simulink model "Noh_Nofusion"  (R2020b)
settings: Solver=FixedStepAuto  StartTime=0.0  StopTime=Inf  FixedStep=0.01  RelTol=1e-3
PostLoadFcn:
  | if any(exist('dsrtsu_mdlpostloadfcn', 'file') ~= 0), dsrtsu_mdlpostloadfcn('Execute', bdroot); end
InitFcn:
  | , if any(exist('rtifpga_mdlclblib', 'file') ~= 0), rtifpga_mdlclblib('Init', bdroot); end,
  | , if any(exist('dsmpb_private', 'file') ~= 0), dsmpb_private('dsmpb_mdlclblib', 'Init', bdroot); end,
undefined symbols (not defined in the file): ACC_TimeGap_DecSetSwt, ACC_TimeGap_IncSetSwt, AccelPedalPosn, AccelPedalPosnVldty, AccelPedlPosnDiagc, AccPedalOverride, ACU_ShiftInProgress, ADAS_Posn_CurLane, AESSwtReq, ALC_SwtReq, BrkPedalSts, CC_ACC_CANCEL_OFFSwt, CC_ACC_CRUISE_OFFSwt, CC_ACC_DecSetSpd_SetSwt, CC_ACC_IncSetSpd_ResuSwt, CC_ACCSwtErr, CharSpd_ms, CSA_NODE, CURRENT_GEAR, CurrentGearValid, DiscIntNeverNeededParam, DrvDoorSts, DrvSBR, DrvTrqReqOvld, ECMACCInterface, ECMRespACC, ELKSwtReq, EngLimpHomeSts, EngSpd, EngState, EngState_PHEV, EngTrqMaxActSpd, EngTrqMinAct, EPS_DrvInpTrqVal_HighReslolution, EPS_FailSts, EPS_LKATorqOvrlDlvd, EPS_LKATorqOvrlDlvdVld, EPS_LKATrqOvlDlvdSts, EPS_SteerMod, EPS_TrqSnsrSts, EQ4_APPINFO, EQ4_LA_ELEM, EQ4_LA_HDR, EQ4_LAP_ELEM, EQ4_LAP_HDR, EQ4_LH_ELEM, EQ4_LH_HDR, EQ4_LRE_ELEM, EQ4_LRE_HDR, ESS_PedSwtReq, ESS_VehSwtReq, FFogLmpSts_F_Pbox, FLWheelDriveDirection, FLWheelSpd, FrntWiprSwtSts, FrntWshrSwtSts, FRWheelDriveDirection, FRWheelSpd, HazardLmpSwtSts, HCU_AccelPedalPosn_Diag ... (+153)
libraries: simulink x132, dsmpblib x27
(part 1 of 14)
PreSaveFcn:
  | , if any(exist('dsmpb_private', 'file') ~= 0), dsmpb_private('dsmpb_mdlclblib', 'PreSave', bdroot); end,
CloseFcn:
  | , if any(exist('dsmpb_private', 'file') ~= 0), dsmpb_private('dsmpb_mdlclblib', 'Close', bdroot); end,
settings Model: RTICANMMDATA=struct('GeneralSetupData',struct('modelroot','D:\ADAS_Store\Project\adas_project','generalsettings',struct('filesettings',struct('destfolder',struct('Name','RTICANMM_FILES','Check',1),'buildfolder',struct('Name','.','Check',1),'AbsDestfolder',struct('Name','D:\ADAS_Store\Project\adas_project\RTICANMM_FILES'),'AbsBuildfolder',struct('Name','D:\ADAS_Store\Project\adas_project'))),'options',struct('addpaths',1,'rmpaths',1,'addtrcexclusion',false,'cannavigator',struct('checkmonitoring',0),'show_usrtrc',0,'use_usrtrc',0),'advanced',struct('options',ones(1,100)),'MPSetup',{{}},'RTI',struct('Type','DSRT','Ver','4.3','Date','02-May-2020'),'modelname','Noh_Nofusion','block','Noh_Nofusion'))  DSRTSU_INTERNAL_RTIFPGA=160  DSMPB_ID_DATA={'104',struct('BlockId','7cff38d8-8644-4a19-b5e4-5036ee6ea8a9','SignalIds',{{'3bbdea8f-b8ec-442d-8749-62bdfef547b6'}}),'1100',struct('BlockId','4ca9a9d8-d3f0-4675-bdb3-98ae5f57268b','SignalIds',{{'65f8c5f7-e719-4be5-a3cd-3d0a65efbc7c','14567e72-e425-4a19-8f08-ff088e7bc1ec','3e363610-daae-4ac2-937f-50da8a805d2e','fbf30fd1-1576-4ae6-a543-209a9facf6d2','e0c202d0-5fb1-4536-b086-d0c57c194c04','c0e2e943-4026-4c35-9218-a0af2d5b6d57','8bfee92f-2cf6-443b-b155-6a457f2e626f','caf28ac8-b870-4c6f-ae52-cb4984ce6abc','2a387729-dd70-441b-bc6e-f3d93104464f','d8bf82ef-2756-4b2f-8a1b-0b3a0445a133','0e21403a-5d1f-447c-bc7f-b58f25cabe9c'}}),'1101',struct('BlockId','d0076d19-96d3-4a18-af19-060cf9157f7a','SignalIds',{{'14858718-5e5f-4783-86cd-d57dc4407506','82655791-0db2-4bf9-9c4e-8101d6dc3df4','e886bc01-ab1a-41e3-b5b9-381a12da1c74','4ac70ee1-afcd-4eba-b446-b68387f1a31e','689c3bac-1bb7-43b0-9971-a5f6a46937d1','02edd042-c75c-428e-8cab-23306c40c90c','cab918fe-db57-43ed-b49c-d58057f13217','ab72ead8-b72e-4302-85f0-2013a3e14f21','1166ec62-eea0-4cb6-ae80-d5b7b4c4a0fa','34e9efe9-6cdc-4a06-9832-9c921a0545b7','1b7d87ae-63cb-4055-a179-c88df6a6f045','ed32b865-3079-4fbe-b7dd-1824d6a55149','7f30ffb5-df1f-4034-bff0-e6d511eebe1b','728925f6-67a6-4dc4-90ab-4b2ad4c99208','c6bc75cb-b181-461a-a367-6900fcbb88bd','8317a6a6-be88-4f57-8078-4578decf736b','48612be6-51f6-4551-8c7e-832774c8bc67','c595a5d8-d15f-4a1e-9efd-3784581641c2','58310f9b-663a-48bf-ac26-6aa723a8a01e','9fd1b362-1098-47fa-bc3e-5a2e8f5c0c2d','451cead1-5ebd-4ac2-ae12-7fbbcf67bb83','9cb3fe7e-65dd-4c40-8287-015a94f704b5','5bf53764-bace-445f-bcc4-fbe30dae6c62','6da7a470-6ef2-4cdb-a51f-4fae12e7471a','60d3bb74-d0fb-48a1-90d5-057b658358a4','ffa9a598-2281-4998-8615-a5ecc23ded37','f9ab87f2-2869-46a8-ab86-8a97089e9558','5064d5d0-55ce-45eb-a3c8-232eacdd7510','e8f543ad-5b2e-4901-86ca-decafb25c62f','1807255d-94a6-48a3-85be-1315832c545a','824ed113-2f14-401d-b956-a14438369d77','260dd518-87ea-4a3e-a881-228651db4719','f5eff198-1af3-4d0e-999d-0c062aab4917','aede5eb3-92b4-4d5d-8021-6c3b3cb83fe8','61c18043-86bd-4be0-a3d8-a1eb1acd2767','42a66cec-6c0c-4b38-bb08-e9ca357fd7a5','56320901-7f7f-449a-abc2-3a4ba0d3d413','9b34d551-a66b-4913-90f3-07aa90245b9a','015840b8-b6ee-4fd1-8636-bb1d9a643f62','c5d51264-f08a-40eb-b0b1-db8cf68002df','711671d4-3b56-48d1-8d4e-8cacf61b19de','d18da288-82ed-49a3-80b3-cf3efb0c0b6d','96ca03ed-5529-4dff-940a-9c6d805b9ee2','176ffabc-6154-4f92-928c-3b9e74565894','4a60be88-e640-4573-bb9c-5438e25d3f5b','54288b0e-bcf5-44a6-9d9a-742a597fbc71','8a2036ac-ec23-4c1d-baf0-14d0d5705fe0'}}),'1102',struct('BlockId','b1879b78-97ae-49bd-be3e-6dd959ea02d7','SignalIds',{{'b184865a-56b8-4642-a9d9-33e216aa1cc7','4f6803c9-4c49-4c0c-bc6a-4fd056ce5919','d43624c1-2988-4cd3-ba78-7b11552dc0b2','0760b15b-d21c-4d21-9c7e-5c6cc820a731','75084567-158f-40fd-b3ae-c40a485083b4','d0e08f80-8df8-4fba-b874-dd6fafcd2bb0','b17d0cf9-4846-48a1-bb2d-a71384e2d6ff','945bc0e0-d807-499a-9365-7adfd37df6fa','58110f9a-7087-4e44-8b20-a6fe297dcb9d','64f52746-4d34-4424-ae18-4dbc9a56c3c7','587e759c-0ed3-4568-8d4e-c2b8e13bca45','b8fe9749-81d7-4d06-8478-96a34fe63437','ebf5961c-0d94-4ce4-b4db-b7b2833f436c','9089f9e4-396a-4d86-8134-6d3956595bad','693d247e-6854-4426-87f7-c7d1ee9d9c13','c20d448c-b801-4195-814c-f833befdaa99','c06ef1b8-55cd-4c64-bdc9-3d9c76d3d8c6','a9470883-42d0-4499-83e8-b60f7ff939b2'}}),'1103',struct('BlockId','40d30207-c21a-4fe9-89b8-31db2ddfcd24','SignalIds',{{'317f5371-3e40-4468-bdfd-f3a914b09fdd','487dc9a7-f215-4486-8edf-23b26ea9e674','56e2ea18-1796-497f-bfc5-34f8a7a00d06','a8fd35e7-70ab-4cf0-bc17-abccda21b043','712b5988-beb7-4069-9325-ac4d1d105b1c','66ba01a0-0e88-4d3a-9ab0-8823bb2078d0','413426c5-cd8c-4ce7-9f02-6918ae7e5a9b','b324e822-3bc5-4738-a954-9bf60ff29b1e','7901db69-3f11-4cf9-a394-c843afd09e88','480f8adf-d9a2-4f97-8224-e59739a90d13','3628ea91-3224-46aa-ab7f-8b572fef6cbe','d84fb504-f908-419d-85e5-1fc1315e5fac','029ee664-06cb-4483-ae91-26f72088f733','37778ae4-2ffb-44fd-a39e-f60bd25d5ad6','f1854a58-8f08-4c6d-9505-83c95ebb36a7','670ec646-6257-4a76-a5d4-ee226aff6fc6','182a7399-08ac-434c-abd3-5469e8d7dc3c','d7a4aba7-220d-44eb-a78e-488b3b0e7d32','f0b7ec55-592a-4cb0-adc7-ca89299845c0','0e6e96cf-5bcb-426b-a6b6-e45252ca00e4','6fe68ad6-5d89-4ea6-a9cc-e00090ddc430','33f16b3a-8526-4185-8ed1-70240d225458','f7e06676-b4f1-4bd4-831a-a554e14d03fb','9f9edd6d-d0a0-4862-92d3-62b44ec6be06'}}),'1104',struct('BlockId','f96afb62-b232-4875-9f16-8cc66b39bf91','SignalIds',{{'60fdcedf-618c-4398-b64e-96a67d35286a','a5abee4c-7192-4b09-b4cb-6b73a01a8785','80a86882-ad5a-461a-9b39-764b3f3b9edb','f2561c9c-264f-4250-ba14-6de6d6d87bfc','5ca34829-1407-46a5-a499-030ccb73446c','b1a0f660-5421-4458-9b14-058e7b19d0a7','3e082988-6105-4757-8f40-1762abe04838','10eebde5-758a-4a7c-9873-029b28255700','b97055ad-af84-4e89-bbec-8426d6ca24a7','02444ee2-6b2a-4c04-bd69-190353a0c672','6b7e1708-e88f-4ff9-b738-fb06481b8050','a61247de-e6d2-4f0d-914d-644a5fac8733','b186f77e-6eeb-4db4-b5e8-55a5ed49ddae','72fb2380-66d9-4408-a4a6-3fdc4c96a441','4b99d9c7-d0fe-4995-8523-0b8e4e0c1a87','993ca2f1-5b4e-4d93-99cb-7f1614d6bccd','d13b3b17-e0b4-40cb-b556-b5fb395c05e3','2b8d32ce-a89a-4bfb-a484-516ae21f5f89'}}),'1105',struct('BlockId','2680f75a-2b29-4fd2-87b5-3498c9e058a6','SignalIds',{{'faa0ae6e-be86-4564-a94c-27f40175599d','4f865cc3-3da2-416a-a28f-e5f9c3832da3','27d74ed4-a669-4b68-bc5c-8acf4c25a9bb','6dbdc5bd-ee8c-480e-9846-77e86fe90609','1cb076e4-082d-4ab9-a5f3-bee85026cdb8','2110b29f-3627-4de3-9efa-dd3d95b1da54','94a8490f-2016-425c-b913-702d8cf19f01','2f9cbf7d-72a1-4bf3-829f-e3c04433bcc1','7f377641-eb9d-4447-8f07-ba1493fdfcbc','32e0a569-e9c5-4c6c-8bcc-77704a185bd1','1a04a7b1-ae91-43b0-927d-b415b38980ab','572d95be-1870-4610-a1b7-429109650953','d91bea2d-baed-4faa-85ed-9673a90f5781','7261506d-eeaa-4777-9a22-f3e4426f086a','10adf570-39c2-4d90-b43f-c59c3584b59b','517bccf7-ae25-4539-b307-30354d195b17','d19821ad-b439-4876-8f19-0734b541c411','df3325a2-916d-48e6-88ff-3bc27aeac87a','22f6a12f-0e34-4c11-b865-9adaabb8b946','66463846-880e-4cdd-9d21-07899b7873a5','07c9a7e7-e28f-4af9-a08a-92ce9b93897a','022c41ff-3ec9-49d1-bfdd-669fbf64d6b6','f28cb986-d944-4ed6-9920-a833a33fef57','804deebe-207b-40c4-8465-d08574e585e9','f3fa9451-9ed3-45ca-88ff-a23189da5307','a157ade1-4d3e-43dc-a7cc-98106a446eca','4b6854fb-31e3-4b06-8063-ea049aa2ba81','62aabf9d-dda7-47f0-85dc-f3ecfe0f445d','c94a70ec-5bac-41e6-aee8-fbef32666ccf','9b83fe42-6781-4ad1-83d7-7c4a17efa7f3','815b8527-3d8f-4145-830e-a0fadbc05b0a','bcdaa839-c535-4875-8ae2-f2aa8b6736eb','674f33aa-9516-4f07-a049-d932dce3789b','a26426b2-6a16-404a-b705-9b68c0dd7dc7','eee14ca8-254f-4116-8e6f-05e0565bedc9','687f108b-366c-4a46-85ac-ac0bcbe55871','b37c0729-9282-4409-ba52-a7f2a4bc6d51','dd0ddc1f-37ff-47ed-8e5f-c2071c6762d6','1b3a4e79-80d6-4094-86f5-78ecd209e112','2232deaf-fd23-43a6-94d6-be881cb58ed4','2a65d406-ac4b-4e2f-ac3c-a87cba00d8b2'}}),'1433',struct('BlockId','94234e05-19a1-4762-bb7b-0b648db02d71','SignalIds',{{'e8c921a0-45c0-4565-a75f-f1538dace8aa','97da14a3-59c2-4f15-9794-12e20298ad37','993ea120-009c-4d58-b833-f257c1bbe946','b0ce32b7-b1b7-4613-8014-a2b096116a3f','d0bc5c4d-081d-493e-bb0f-3880de0830f4','f577c16d-4f84-464d-bc22-208daba2c996','dd8d90c9-db10-4aee-8f78-aab1d2b07a4d','786cc827-4d3f-4751-8aac-002e08b48fca','3cc83904-5789-4284-8d89-c149abb24041','066cabaf-b5cf-4a22-a486-8d7bf34a30a5','14c931a2-4f8a-4067-a3ab-e1ebb5f58bae','3318169c-4586-48c4-8457-857db8f36c39','afa8f609-89b6-4cf2-8b3b-67301da0d077','db3dccf0-ac50-421f-a652-6186d40f7434','98c83b7e-8f23-48c4-966e-4a54d21b7757','42747761-adf1-4162-a5eb-1d7b1815f06f','f4026a07-0643-41fe-ac5d-129eb617d3bb','a806bbcd-b881-4618-9bc2-15c80f567ed0','dd8efa00-8fe6-472b-b374-365213651d88','17e98c86-4a76-41dc-b5a1-c6f316a60d0d','f2c4471e-757c-4a82-8024-244d60e4eae0','0baafb07-de45-4b4b-a0af-fc29d6b90e2f','7deeb15d-c086-41bc-a56a-2c4b692487f1','2b0e0941-927e-4c06-ab5e-2abe3916fc55','5584579c-2ab8-4aaf-b9f9-629067beb1d1','7936e867-fe88-4af5-b973-84858e665a13','c57a407d-b218-42f5-8846-438e73728874','90881888-af9a-4cc4-a1ae-0ecda3135b42','ec3687ed-f2c9-4806-8c7e-30e4660968c6','d4c236ae-2feb-4f6c-9bb1-7b97a6ed9825','8eea8e37-c910-42dc-a602-5540f6a14377','e9ac2b78-f63e-4fc9-95d9-b858b89e45a9','abb40779-4b61-4ab4-bd71-3a821b717804','7fb27904-ab07-458c-959e-9464df60189e','cdef6a3f-3536-4e6e-a717-ef2141c6625b','7766ce8f-4903-4070-8e33-31e989b0c27b','5ed6d31b-ff27-45e5-80f1-63a2314d3977','703c0186-0353-48e4-9ebe-c7e62be1761c','90e2d2bf-e9a2-4e62-963d-e2118c02d3f0','159e3cc7-cce6-4e38-bcaa-fd58f86ac572','7b2e5dd3-de8c-4c77-a57b-9641b9f21836','0c7c6a3d-5efc-4a2c-8d24-02cdd2042006','379efa5b-3a39-4d46-80ca-c859689c2b8e','f549e28d-aeef-4011-b98d-621e8c092949','a26c273e-3059-4d1c-9ca1-60671908df44','8cfd88fd-e834-4fb3-b7a9-6a942acc2f0d','f5cddd7a-0da6-4742-9f4c-10fbd2b3f6f7','8a39439b-2bf1-4344-9b5f-42eb278b8376','8ccf14d9-6c5a-4163-9001-5177855509b8','f5b88dff-d83a-495f-92eb-bece265ce1e6','9dc0ae1f-9d6d-46e8-8842-1ad9d25be10e','5a77b2d3-cbf8-4b9a-a1aa-23d3a249b441','3bcf1e6e-1d26-4903-a127-764aed52a8c4'}}),'1528',struct('BlockId','d10b6a7e-e28c-4d43-9d3f-8d5c2e8198e6','SignalIds',{{'d97805f0-7d23-4e28-bf97-3f26e24bb340'}}),'185',struct('BlockId','027e024d-1595-40f1-91cc-6eabca2a1c6c','SignalIds',{{'af9ca425-4598-4529-ae3a-7e01afab32e2','5b6a4c10-dcc5-4361-b694-7f13522380cd','328b1ae8-99c0-4358-aa60-26f71449921d','56877a5e-a28c-460d-b602-6169d6e3ea29','ff774db8-82bf-4d5d-af96-834818f3b92b','454bb863-e562-4923-b300-500615260782','a069b205-7781-45e2-8fc6-dbc7346dd223','cdcb80d6-e457-4c10-893c-2087872783e0','6b56bd7e-1102-406b-8d36-39d13718a3c9','254c0b29-47ad-419c-85d7-e9515a2bbc5a','a6c2ea10-dbc8-4b2d-879f-4465f4c97ead','84746e2e-380b-4ef4-a4ee-2f1341934cbc','8a1fcb45-6acd-44a7-ab31-c33169900c5c','1bb09bca-435b-416b-bf20-aa9f8dc89494','d5011b75-efa1-42d0-986e-b3cd336946c1','c50ad309-eea6-40fb-8bb2-c8ca0fd215a4','85488a99-7b3a-49f7-9866-9335aff8292f','1b523a6a-dad5-4454-a82b-427cdad5527a','e3668b27-7252-480d-9bc0-b61d6693a235','cdb3337a-376c-4be9-b00d-011122b2f594','9e493416-6a03-4c36-af69-81d560cc7c26','c974d250-90a0-4162-a8f3-f2bd83b95395','d04338fd-2c1d-44c1-83ef-f5a12be17f66','6b9ced49-9cb6-4a69-955c-e404182980a0','b674ae42-370f-4555-9541-dc621716dd61','9984a409-650d-4478-bb6d-7bc56841d6f8','13af6717-7a51-4ea3-9a56-75b6a52376f8','4e0778bb-f83f-41f0-8d20-f78f6ce92b3e','4d28c29b-7e1a-40e1-911b-92780d01b3e7','c8c10f1a-0381-40aa-bfa3-55e0f65f03f7','6ff69308-3cf4-4357-8220-b029ad8d6e5f','86c10f87-d80c-46c7-8547-d972b3c72066','58824a37-65e2-44b2-8ecb-9a3ceea53242','4cc9ab58-e370-427c-a1eb-3f534084f586','46028ab2-a792-422a-8188-bf88d7b32cca','2620c9ac-a16e-43f2-9cd2-303aa9482609','8d5f6dfd-c403-466d-afb4-029409fb64c9','ab18518f-d5cc-458a-bf16-a266b29bb816','c447b944-9d82-4738-96e7-e805931a61d6','4648cb0f-e4b2-4d8b-b4ae-78edeaf07ecb','0d5f2b7d-ffc7-4c2e-9926-08fc4b38d8d3','cb305857-3bab-4ab9-a512-13b5cf4c3611','882887ab-9221-48c3-aece-5f62605b07cf','c1ed5e22-0d96-4be4-a264-775bdc9289d8','8dfcd5b3-3f6b-47fe-bfd7-360309192973','2f5b9f31-e322-4e9e-91ff-2b792e269494','9c83eb90-5594-4393-b68c-76083cfd2368','c3c853c5-575c-497a-88e3-9bdc8151587f','39bc0fb2-c156-4fd6-823c-d838e9b415bb','11e4d06d-1866-46fe-9d96-515f20b3a166','d28af3ed-bcc6-4c20-a67e-4c6edc30615e','300473aa-186b-431e-aa09-bcef650b1d10','525ba979-9845-41f3-bb88-9301b545eaf8','9086135b-c809-4b03-a647-5c809e7976bc','fb7747ea-026f-4131-b788-d0080cc2d781','1bbce54c-3b61-4bd8-b70f-63a014235e41','34aac6cc-aabc-487f-931d-6f59ca2848ff','7c379fbd-fe17-4d8e-92dc-a558699f97c5','01f6d5e1-fa78-4d82-8816-5e72f37309b9','bd593841-debd-411f-b281-21f285214c62','530633ac-2fce-4482-8f6f-36f96f2279e6','e2ad15e5-d508-4424-abd5-058f42272fb0','2e869d70-f0f3-4c63-b867-fc338524c6c1','c39af9fa-b12d-4dda-8908-43a002b021e4','f55a134e-cd44-411f-b8d1-d5384f7d9bbd','44733f61-e0a1-4296-a072-449191a0d7c2','236717fe-2e36-4baa-ae42-fa0a21285d60','b93dfc7f-fe30-44d5-8a64-20ef4cbe3e05','77aabc39-1faa-4cfd-bbb3-56d44336e653','842bfad2-8751-4e0f-ba9a-49bc3ec717bb','2e40a366-aaa2-445f-9cd4-d7db11225b25','b20b6a0f-27c5-4321-8600-7a46806b1889','ff122335-ef39-420e-951d-0bd347c0bbe8','858aacba-ed21-4fda-971e-365f2a3bd691','dd61c21e-cb19-499c-9c1d-430d92200507','28a1d6e6-5e07-4a7f-a715-f9b360cdb100','ad1e1c87-681c-4047-ba6b-7e601469f270','0391655a-ff16-4302-9c07-65d31e4e455b','b0ef2e95-a16d-480a-808d-79c9fd551dd8','ffb54581-e06a-4a0a-999a-186bbc24b3d0','0012874c-e9f2-4528-a1e2-357d36894825','9b0be146-16d2-49ca-87c4-d3b216fa8a7e','4b3dec22-ab7a-451b-8ed8-67b44c9e403a','1e2cd59d-2718-44e9-b09e-60f7a9896aa1','229c0dc1-1a35-41ad-8040-9a87d0112535','aa2beafd-4457-4ccf-9ba1-dc93627b92f7','4c9b48dc-2935-4b3a-b559-253566d53f0e','2932469e-7c4e-4f7f-ba8d-87e146d3f32b','5af95647-4500-4523-b254-1acc3d27f61c','0ee114be-31bd-4e49-99d8-83f6aafc12c4','e421cce4-1282-4497-b07d-0fef94a7301b','5e0791f7-f6b7-4bcd-8cad-4d44dedffe48','17b877a3-82f4-42ac-a246-510955e73fc7','a3aa4786-486c-4baf-9e43-ba20b0f728b9','d190471a-81d4-4fb1-a2c4-6343843b1016','cfed4979-3935-4876-bc26-9f5361a4d7e6','fe01ece9-a60f-4854-a4a1-7c7ba81dafee','3d6a6da0-107d-48fe-88b1-1d4261408128','7667d7db-dcba-4862-8709-e6592637f797','2768002a-5121-4ccb-9348-6388c040144f','ec34afc5-758f-4e7a-9e48-a30da6158a05','0fc73188-500e-4129-b6d7-621b3ab9d0c2'}}),'190',struct('BlockId','743152e8-9ac7-4ad5-8bcb-62bd33860f51','SignalIds',{{'cd70d485-29b0-4608-acab-f9a0ad4ae544'}}),'2',struct('BlockId','834cc0d5-34e7-46b6-81a3-1dcd68231e94','SignalIds',{{'6fef6530-40cf-4af2-966e-1dd99a7db263','8cde6f6f-cbd6-49da-bf0d-2b1810a2f3f0','221dad7c-d002-448c-a0f9-58b1c04b1f3c','b8525d83-c558-4b75-a1e4-1d67d733ed8b','2be87e7b-74d9-47bb-9903-4bfd77754f53','c9f3fd7e-8135-4b39-b6d7-770c409665ed','4702f466-3408-44af-8014-ddbc449026cf','f2a675fe-18cd-4f9f-b14c-0423a592d937','9581e41a-39fa-4f6f-a3f0-97af6d21fdc4','e4bd4dad-ee04-4c19-9d54-cb67c246147b','941a1b62-d594-4634-87b3-ab1089bc0a3e','b2ca4db9-33cd-42e9-8506-7bfa5542326f','dd4f90c3-e069-47b8-a07a-200f1c201139','b7f618d6-3dd1-46ec-8cb8-e0444cdf2ff8','113b0bd8-e176-471f-b570-1f2540c1d312','462ab9d4-6afc-4817-8085-26039ef68426','aa53af52-033b-4610-b93b-fe3e7eece305','6cc13e12-629f-433d-9603-bd6de1e7c25c','504f509c-8beb-49d4-ba8b-8c53242d288c','4b8ac33a-ecb9-439d-9992-db75439c2ca9','67e3a30a-5548-49d3-92b7-c219ef59e1c4','b89e8d70-bda6-4353-a3ae-62619d5ada82','dceabcca-c3af-46af-bcbd-c666f0f7bc5c','df238af6-7873-4e5b-8368-8ea3dc21d0a2','7ebfac03-ac16-4e22-bc27-abe381f0c5ca','7f822ce1-daad-4675-8882-0aee4907823e','141ce932-0e23-41bd-afba-086e17f31757','4d75ad82-2038-4c91-bb5a-2b06d2ea7f3f','89785920-ae71-47a4-baaa-3ed970aacc47','d7e8ff71-3f36-4a4c-8a3e-7459b2eee384','c5737a51-de96-4e9d-b4e7-e59e330bb75c','596b8901-f9e7-4c42-8df6-984a90c5ccee','ac8e446f-949f-4550-8cb2-44382d50069d'}}),'221',struct('BlockId','9717df85-bcfc-49b8-a662-c8e164f93e64','SignalIds',{{'98218185-603e-4cfe-b8dd-87d73af7d6c1','0ae18e67-df76-4ab9-80ac-08b5cafae14a','93e36128-dc12-45e1-879e-1d03dab6f3fe','60be3b9b-cfbc-4439-9d52-59c083c9d5da','ce4b33a7-66e6-4025-ad5d-457152d62728','47a10254-f6c9-4020-bade-5da6bfaba0bf','4028a858-46fc-4356-9e2d-568c8c8d5185','92e9d05b-648c-4753-9092-7efc6706eae4','2bbcc664-c65c-45c0-b39c-6ea8c98967fa','2e8dabbc-679d-4ccb-849d-2087c0f92e6a','e06e10c2-8017-4579-b849-8d941b033611','5269ea5b-c8ac-4336-98b2-3b21ee315d23','d2a52c76-af8c-4439-8ef6-7b1d2f83305f','268705b8-dbbb-4302-a8e9-3f328f1bcfbb','5e66467a-52fc-49b5-99b3-20ff2e18aa45','a45fc991-8e4e-4c8a-976f-36925d9b7a31','fc407165-2dc4-407b-9ced-2c66288cb330','e7399825-9566-4d29-b564-c1d9af99436c','324bbb31-6a7d-449f-9ba7-a52ec84408a4','55a4bc7b-f7a6-44c5-afd8-1af865882ea8','261aacaf-414d-4645-9744-1e5fb6eea559','1b993f21-9c8a-4541-8356-bce3bf8b598d','5b233cb4-a194-484e-aebb-07eca2b645cd','7013e9be-983b-4d0a-b921-1bdde5140462','07cf7efb-44d5-4609-bf91-9b6a73cdde14','fd74568c-b72e-4b34-8d22-5fa171842560','dbb6928e-c632-4ebe-8fc8-79609d9fcbc6','bcb57694-ce72-4fc3-9bf7-3deef866cf49','e3fb6b0a-adc9-4f9b-986d-51694bf4d55c','3ca1c8cd-3546-4e20-a829-927678026f67','b650e98e-6faa-42bd-970a-366b863a238b','54c7e6bf-25f1-4ce0-ae9a-ae2ce10a926c','223a6c20-f064-490b-b70f-cfd0a8487db3','d5257b18-6a4b-4ed8-baa1-33a625deeb69','0cd3b500-ee4a-421b-b5f2-673934e9ed1d','b70af485-7820-42ba-930b-7fce961d7c71','a41ebe10-051a-4453-a09f-b91c40e454bd','8d19cc93-71a5-44d2-8681-4483879a4487','f81902e1-f5c1-47c6-b5c6-a13dda42f95e','cb3a6e21-59a3-4930-a05b-e5dd559cd7c5','bd801981-6b71-432d-b7e7-a32e625948a8','4bfc8570-5612-4bff-b1a7-6a72cb419248','b7c0e552-9857-4fd2-956c-81a8842b765f','94aa017d-7e68-4b88-821f-85ce4d1ef8a8','a3ee68b8-54a6-4169-8089-1d4d226e997c','3a0fba51-8047-4949-a4ef-5012e451e1e5','409c24d4-99b9-41de-9e44-7afd0917e5fd','83bab7c9-7a4d-4145-a489-31e7a45e06ce','7e1593a2-2f92-47de-b4da-13b6a040434a','6d1a8d38-3f26-42e9-a24c-574b4e61b6ca','17a9bce9-b7fa-44b6-87ab-af45e1691c0c','d78c8f7c-42cb-42c7-aa7a-f7cc863310cf','eac6c7e9-474a-46dc-a464-7be55b2efb83','41630e37-ad8c-4986-8ab8-339c549466ad','00890894-e1ff-43d3-acd5-e44d2f50b47d','db8a4397-9d7f-431c-b2a1-db715f9d0f84','ca7a6001-81b7-46b9-aca1-f7bbe4928958','01ff805f-5202-4eb6-a5be-f7b65966125c','2dbeb2f9-185d-465f-87f7-b63ad955f1ad','0a1977ac-2488-4528-99f0-0b1c82e84f33','0994b021-cd20-4c63-a6a8-a42bb3614797','2686ebc6-abab-4acf-9441-dade5e1bbcfc','7bc5d66c-74bb-4814-a4cb-9f6bd9f34925','e024091a-ebcc-442a-8da9-9e6d9588439e','c1916b73-542b-409e-80ac-a4299c749a69','5e05ffd7-18c9-4195-adf6-aa8e874a9ac0','4193a004-68ad-47e9-b796-0c54da424369','f5799e86-f50b-4574-ae26-5dbae8af9391','e7728ca7-f8c4-4fd1-a24b-2bdbac0174a8','151b3bf5-7fec-4d57-99dc-3ab84986106c','17ebd3e0-fd97-4f11-8c4b-aa9ae55f55db','5a4a7d70-8c87-4ef1-abd7-1b9a3a823da5','0012e72b-7773-4b89-a60d-b04569bfd203','bf3f289f-87c0-4201-9c19-e93e6d6681ca','a5d29572-8266-4dfe-98d0-c8ce36c56e70','e4b259ce-263c-4fb5-8a15-be6db67a3c9b','78a4a82b-821b-4a70-905f-a02bad9ea87b','22914ecc-c2d6-4c2a-9888-63dc66ff5d49','e8eec08b-4b86-4094-8f75-c1efece1608a','b6301d68-59ac-4819-bc08-0069381b0e44','3808d26f-fbc4-4df5-bf3a-f6fb71ad741d','0c7d15b6-698e-40ab-b0a1-8c0942cafd35','517bdcc9-7989-466a-8333-bdce3f05bbcd','adeaa512-e2a3-47b2-b97d-46754f529463','3f0e7aee-1ccb-4163-bd9c-b4b3cddc4d1a','701225a3-1260-45ec-98c7-19e4cc14de3d','90777c50-6ade-4ce1-8bf6-ea9bd8814c97','55d79536-57c5-4c5f-8f8f-b10a1bbc1c72','418a5e1c-09e1-4ad8-a4f7-117d51134268','d81b4e32-cfeb-4b32-82a1-b3ed4a1e2306','48f5decf-67ca-4aa0-865c-0cc27b4d829c','a8f75cf2-e84b-4091-9f0b-311e40b38a0c','d34f1bed-f2ef-46a1-b17c-14676bd34d43','6a6836c5-df25-433f-bd7b-f06223bd88a6','a56286d3-3ffb-4b57-ad38-12774465bd47','1e5f4f7d-bea2-4ca6-a880-12464806f91f','70bff75d-907f-4d0a-8437-e9ae070dd089','0e270762-ea89-461c-a4b4-1962f44588db','701c306e-8378-4067-ba6d-b44e8713e082','eb1b602b-4471-427d-b80a-81767a3680ab','3e652b9a-337b-49f9-a534-b580c5fa8842','8b8316bd-73c1-4eaa-8de2-8d90ee05edfe'}}),'226',struct('BlockId','4ca5ff50-ede6-486e-aae6-243c5a029b67','SignalIds',{{'da8de703-dd1e-4566-9b8d-ab888149e396'}}),'2415',struct('BlockId','35307dd6-2333-48b7-9c51-40bc5881f077','SignalIds',{{'8f21a055-1119-480d-bfb3-4aada2b9e621','13040f22-6f3b-4259-b31c-d9c82d97f29e','c219f4b1-6d8d-4cc5-a7cb-ad8e2a5c3fc0','7ea8586f-d115-434c-8dbc-541c7c0338f6','e688c2ac-5ab4-40d0-b520-0934e0380d10'}}),'2521',struct('BlockId','fd219436-0644-472f-8d2a-6a4ad77c9484','SignalIds',{{'10d28b96-2528-49e7-b3c9-39b72b16eccf'}}),'2522',struct('BlockId','79ecf02b-efee-48cb-80b3-e2365e9aa7e2','SignalIds',{{'768929e9-c6ae-4ab6-904c-312e7f4ecf37'}}),'2528',struct('BlockId','e465ec9c-2cd4-4e00-84f2-0bcb180c04df','SignalIds',{{'98ba9243-8cfe-4110-86b7-625d0ce95712','01545a84-5b7d-4ea3-9dda-fa144c4e31b8','4ecfd1d2-c628-4bfa-b3fc-64b927cc045a','76ebd2b2-2f0e-4651-80f3-294187615cbe','5c5ac8a3-d27c-4601-9b54-77ac4b8a3872'}}),'2535',struct('BlockId','ad2f62a7-1ac2-49d2-b87a-6930b7097689','SignalIds',{{'cd925257-0859-4358-87a6-b6d31879bfa4','2658ca35-8371-4ca6-a336-d22da8a7c2d3','acc8f4d2-06f4-4bda-89d3-75b6f7795f7e','73b18197-58a4-494c-976c-c53b5b1c1cb2','7814e992-6f47-4729-a5fa-fed9fa86bc04','68736755-59b7-4be2-bfc1-afcea2aa567c','fb6593e8-b3b0-45c0-a2b9-c8b62125e5de','75a343b2-e985-4a02-b4e6-0759ceee8c41','41c14a3c-337d-446c-9136-f7d2fc4fc4b1','410787e7-a9e6-436c-8bf9-13641b0c39a3','57db9705-e832-4f0d-927b-5300cbfb20f3','dcbdd59a-3bac-443f-8bab-3cfeb176e1a2','285c20f5-b8bb-4aa8-9711-aee099e2dd9a','5aae0ab9-0f48-47dc-9ece-fd722a2b878c','83393fee-1525-4c93-ab15-29a4e7b3995b','d8d1e245-3c7d-496a-b276-59307fb137bc','edd7f72d-ac8f-4cfd-aa20-fee37a33267d','84b3ec0d-45d4-4bb0-9cb0-1ec1c23699fc','a15064e5-4e46-4b5a-a01e-538923793d44','a6348a9e-dcc6-41dd-9d3f-def4a722083b','a6b58e2b-9b08-49eb-8ace-55dbd100ba63','f5a5b37b-dcf9-4b64-8b74-e159cf22970c','17405164-83f5-4d56-8739-67f9a591342b','356898d0-cced-47d6-b19e-47e223be16fa','9e3fd182-f105-406a-88f8-135c535a844f','7fb1c530-7736-47e5-8495-86a7ec5b9c0a','75eb5e12-df5a-48be-a668-13eb6b6e4778','1cf2c9da-b64a-4dd4-a0e5-18b04bd66557','950d7faa-9895-440b-9071-d124b053260d','e1a1f4e8-ec89-43d6-aa7e-19ecb28466b3','1eb94fd4-7870-411c-88bb-ce568836db9b','240715e1-1f28-4765-b796-bf040b2ee043','c4101dc1-7329-410e-8249-0ce4ceb4c46b','69304e72-8570-4416-8297-2eaed2dad6b5','0c38714b-db74-40f8-8c94-28ccbd1c6a9d','58d45120-bf3f-47eb-b84b-82a5bcf7dc5d','0d096dd9-9fc8-4620-b42c-128713491fe3','fcf29bba-ec00-482d-852b-f43db5311a4d','6d60b787-0b8f-448d-ac55-9ebf11ee196e','caf962e1-e571-48e0-a7eb-c63d321de88f','9e572d55-e747-4c83-a0e2-2586c340d8e6','420ac08e-c40a-4feb-9266-af30a4b8e457','8e357133-4832-4832-b644-e8775a73b750','be63c4f5-129a-4a6c-9758-c28df814d458','d14d4f5b-905d-46e6-a2d8-66f646ed181a','f3a2c5ce-07c8-475a-b926-ef09c5705d4c','2d111d62-eecc-4aa2-9213-22f4e55dcfc2','309db132-f42d-44d3-8f0a-6487e29852e6','384c8f4a-40ca-4346-b98a-6bbb098f5099','bea34073-4315-413c-b7eb-1c6823db2849','46a5f4ed-1b7c-4af4-a3de-e0d6af5b039d','5fe52087-45f4-4442-be81-7d5008a6b7a5','6bfe6bcb-9380-4b9d-8351-758885bfd8c5','5c432e4c-4164-4158-9c37-f14d224e1534','2def45b5-d5ea-4f06-b598-1e087f4c5655','7a49fffa-c0fb-4410-8422-782dd9fa454e','d77e6f5d-44de-45ff-950d-c2b268f2fbf9','1be1b74c-b41a-4dff-b990-523d27e0e718','83afe428-a502-4e48-b6bc-09a185ce1d2e','f1a49aee-1791-4b08-a719-3792986db135','ebf0d9af-e782-4a1d-b81e-456dae42ae28','970a8a88-9601-463b-86c3-d4d85b0c463e','f92d9bee-c239-44b0-8659-8d09a9a3e296','04346b94-cfa2-4297-92a8-acd7d88d4604','da0726b6-42d2-44d7-b030-8e6ef12158cb','0e59f3f3-96b2-4ebd-b397-f9662d5f9f6d','cbeba8f5-e4cc-44c4-abdf-f8054d54378a','64811081-2ee8-4852-ae0c-fce97cd77332','74cf2aef-849b-4c3e-bb17-71c3eb6e469c','0e2c6793-d409-4c78-93be-1b76c3ebe6df','2703b39e-8f20-41fb-8841-c44abac3f832','3534cd5c-f716-4848-87e9-552c8402a8cf','a620d3b5-6ab1-48be-b5bd-ccfad551764d','ad052aed-1591-4f84-94b2-8a4c104ac07a','28c70492-8512-4b5e-ad34-c96ae0aad716','6c15422b-22d7-494a-9721-427021e9e7f7','a0daf83e-de60-40d5-b18d-edc0f7344c58','82ed01b3-8a8e-4e0a-af81-96a6e2021128','3e7dc4e2-6e99-4513-ad94-9c4058f0a134','509f6a8e-a23f-49a1-a554-d6065e1d36ed','12faa9bc-ef12-4c6b-a20b-ee4ede9594c8','d44296d9-2a8d-4ab4-9165-9fa27431d319','48193746-35be-47c0-a7af-1f9a5f4b4966','6584daa2-3358-43b1-ab8b-d33147024b5c','125b099a-5718-441d-b57b-ede4611696d1','1f1a9469-842c-4e87-8ca7-04ca5019acb3','9aac7f63-df6e-4305-9b9b-f352fd0629d1','619c7752-e196-4860-99d9-7d2e7e8c0428','49f19339-add3-4ddd-8f8e-e496ebe3b0a7','c685b0f4-0206-4ae0-bf69-ec657bde6e79','ff932246-70ac-48b2-8ffd-bcfc69988240','b6ec8999-5e68-4906-a17b-b6f3b9ff77fc','d79ca0b2-448d-4e34-8294-da465416a3c3','0d5f9f58-2f06-4be2-a4af-46ddc10da9f0','50a564ce-ce96-4fac-9f6b-5334393e01e6','3659a00f-331e-4cda-9cbf-5fad77b5ecb1','327bab3b-c567-4f39-80c8-1fc3d9e363fe','f4a19413-ad39-4333-ab3d-82b40d69e497','59f5adba-d0e4-43cc-a98e-7ea37df318ee','3692ae8e-aa25-4989-9d07-9dd685717f47','1f53b80c-8e65-402c-94b9-2aa912a80a0a','5c019277-1140-4322-b654-f27260a50f1b','0894358c-8567-40f6-9205-6f4339e7f0ca','f944067f-46b9-4220-ad5b-2068f3a61e62','65d74f68-2ee2-46ca-ac30-b6fb6fe0543d','b10b68cb-6294-40c1-b949-b85b3d65152f','3786ecf3-8ea3-4f8a-b40a-e42d9a3008eb','123f581d-b8ad-4aeb-a5d8-e2ee907d047f','fb9ac52a-4e69-4a00-9a7f-bb6f1d6a4d0b','2479a9ea-4e21-4669-8bfd-1093ba6348da','f784fc7d-3d9b-436e-9f06-06fd2db52b94','d8725743-d40f-45db-800f-0fe8aedeebe0','721f632e-85c0-46ed-90f6-d2d944e7c82e','a0001513-c811-49de-a371-1ea07c83aa21','bab16ae1-bf5c-4585-ae7f-d67998b53d82','678e7d85-af5e-4e72-90b9-13714f45994d','32e467b9-bea3-4452-9b08-374009c49f1e','a74cd9c9-544d-4bb8-a631-c20a5185fc40','082f9a48-235a-4e88-b51e-06de1c04a3f2','73d0242a-42d8-46e0-81ea-9146be6c93eb','24b064f7-54fa-488f-96f0-64e7b61e1c45','7d0ed7e9-643e-4b67-97b5-e52e5f097150','2dd246a1-228c-4e5d-87d4-151ed62d2363','96b4dda1-a2c5-401d-a44d-1356646217a0','d8ae40ed-b381-4325-bf66-53476f446fd6','c5be2f42-6127-4519-a669-5e73e18a7b15','c9cf6659-0c60-45d7-9d96-6d42cbb9d857','8b7b5046-f007-4383-8af4-90c5c81e4452','2cfc0059-8463-4703-8d88-c1e49ae6c2b3','3b26352f-728b-44ce-8293-226322747040','774596e5-9759-491f-b3e0-ce2f450484b7','4c5b8886-d7fb-4a32-97d6-d776ce575f1d','c3b4ef48-dbea-475a-badd-5fa7c6636e91','bef65f17-d534-431a-a5c9-a01c2ff6e969','5d8bd3ac-515a-42ff-953f-9355f6a75edc','056cfd92-380d-4677-8a7a-eb276b3d5ec6','4904b07c-b27a-4e2a-a0f2-70deca69169b','1ad3c7fb-38e0-49bb-acb5-b02af1bc7f08','837569fa-2973-4783-8a3d-e30ed3af6bca','2265b357-38fd-4ec3-9d62-36fb325d8c47','af6c5e6e-a3fd-40cd-96da-58a3246828f0','6af32651-f06f-408e-8b16-93539748053f','76d23fef-41e3-4d8e-ac0b-f2bc54b90e0e','f595e093-e25d-4df5-8005-7922a868ba3c','1c260597-6f78-4a65-8c06-8699ae9be719','bb724f19-e62d-482c-b6db-8d945c4f3a2e','772267df-5616-4ec7-a5e0-5a1513908be2','48768843-dc46-4388-845f-c02b30d3b484','76f98ae2-bd8c-476c-aec5-3e6f419654f0','091ef3c2-18ff-4ad5-9ffc-400cb7ce2432','ba14d8f6-0211-4564-a506-edd28280e0dc','30369aaa-1be5-425f-8398-fcdf470fa5a9','a72f7ed2-1788-434c-93bd-1c63435340e0','d8f032ac-69ea-4465-926a-77853104efcc','b21103b1-fa82-4643-973d-bd03f5129a1d','7d085cfc-2b6c-4498-8517-9b98684d89d2','0ea0cae4-80cd-477b-ad97-d9e6c140eda7','67c5d2ec-daaf-4f92-89f3-dd7e1faa008f','c3a63cf5-9f31-4675-9c8d-7754feecb04d','ccdafe49-6453-4dc1-9be6-c8ac5c536e9d','0fe66ab8-df1e-43fc-b480-6e4620c78ec7','42996598-28a0-4483-a6da-559d66517792','ba81417b-7693-4365-af50-cd6fdd47a034','b85f49df-ef4e-42e9-9a59-5acacc60d994','4dc59843-d12c-4f43-8c8c-e82316580545','330902f9-fc74-4f84-95c5-a844659c3760','fddc2817-af9c-4f1f-aadb-63f2046e7c50','e0c691f3-29e9-49d2-a1f9-3e5ab823e43a','8cc9a661-8ad9-45da-8acb-0101b9fdf4fc','1bf5362d-818d-4bd9-ad1d-893b3fcb67e6','b143eba8-600e-455e-884c-0b3464c60d1a','fe420568-d998-424c-94df-daf226983f4e','998bf25a-367f-4936-be53-bdfc395e05c8','7cab9ef5-96a3-4955-912f-31a68b4601b8','27535f1d-30de-4449-852f-f2fdbc0a2966','069ac587-076b-41c6-9d25-1a88a923f2fe','68e2d4a7-6bab-4caa-9367-5b2951356446','b4e37b4b-06b2-4a04-a7c5-f7b9535b22ee','ab6d430a-7f1d-41ff-9eda-005d809c4e0c','d7ff07d2-cfb9-4f8e-868a-0e8ff3307a0c','777e9fd3-c50b-497c-bc33-1dd4b0e3348d','c99202e5-c997-4fad-a7ce-24e6b73892cd','d6a35d10-68eb-4577-bfd0-86a25f30c2d1','a3671ff8-2949-4a8f-bf26-37039f6ac98d','efdeee0d-c114-4278-8470-808efb5a236d','d2cc0d82-b571-4bb3-b5fe-f24f60b726b4','12566363-8264-41be-9124-59e2087eae19','116b87ff-282b-49ca-b4fc-55b033882194','16b68f71-a692-422d-9adc-ac3dfb39df0e','82b70e70-d6f6-4cc0-8580-ed84e8237dd3','0685e375-8836-418c-b63c-43c53df32502','646a7abf-c9db-4df5-a714-6368c25ba11e','6f8016b7-39ce-4f99-948f-3c78d0ee26db','f5cf218a-ae07-4635-aa06-c62973087a65','93471357-d658-4eba-bfb6-4491df60f0e8','b4739e0c-3de5-40f7-9e0e-36d42b0b9fd5','aef79823-1456-4e98-8ca2-4ede7a1db2f4','280b48dc-2a12-4d4f-8664-a0ac113f4ede','933a1f88-55a5-4bb2-b35b-2a908259f0fb','fd4d75db-ae51-449f-862e-f997cc124349','e65a73c7-c755-4bf4-8399-a507d6bd2cab','5f85babf-21c8-4c9b-8047-73b25c827d97','eda136ea-d6af-494c-b8fc-8f86edeb4714','dfb95d6e-2927-4ff9-8a5c-bedd18d56cfe','0e87a811-7f93-4b11-b487-2bfc4fa25a34','20a54ea9-aea5-4abe-8786-190dfdc39cec','39a8262d-7b44-4f6b-910e-2ffc5619e8b1','e73a79d4-d743-4b1d-9f82-343fa554e380','712969b8-edd0-49a4-86ae-03840392a633','49203373-3c2d-4721-a088-30fc27fd027b','ed6e9c10-4c5f-408a-88fb-4c0822d82eb9','81f87884-233e-4c1b-8cf6-84846c63024b','9354702a-2ca5-4682-99dc-668d815d2a68','e3958898-bc44-4f5e-9312-dcd2942555d8','1bd45eeb-6844-41a5-9539-6097e8349a91','9cf0a44d-4678-463a-b27f-62085cd0c199','880e6bb1-ef93-4982-a3af-58ab619a52f1','26eb93ff-60d5-4a3d-961d-80dae889065a','f7ffe4e1-d544-41fb-82a6-bc4fcb4c80b3','7c8aabb4-4481-4c42-80aa-e51456b6a09f','726e5e91-e4fc-4e64-b88a-059580e035df','af038bfd-a2ee-410b-a98f-bb28d7f58d15','890a1abc-ec68-4fa7-8b3c-0464e3aef7c7','56e10565-4b0c-4740-aa7a-a15f25ee5493','e956eb7e-5420-4545-bf88-ae8030774f9a','3fbb9942-2abc-4f80-bed3-275059c3654e','eaa76a4f-9181-4baf-a67a-6db015e52f38','430677fb-8e5e-4f61-b449-967b3a66d429','c6b39610-7adc-4274-b1fe-b4a58de15c7a','aa7033a9-e422-4b9a-8159-19f5912f05cf','4203db3a-4162-42c6-a72a-e8a2b382ce75','7c9b4fb5-f787-4acc-ba18-6f2aba28e5cb','a7e316c0-e682-4a20-9fd7-74c03bd249e4','58da85b7-0e4a-497c-9fd4-c452ae053325','9eb84c81-1936-4a5c-8b29-26c862863575','e1a54e31-e187-4187-8b3e-13c6a485b0bd','dfec769d-98e4-4998-a532-a17032011462','b367ae17-0fc2-4fb9-b499-871a610b91a1','e1297479-6463-414b-ab07-01294a2b51e3','a2f89142-9095-4d40-bf0a-a4f63496f233','8ec7894d-84e3-43ed-8022-5fda62691d22','30fd786a-008c-4a33-b89d-0c71dd14dcc2','20d3cd3b-4731-4cee-a00b-9b5ddde222fe','f6661d48-929b-4713-a0bd-a2820bc2fb60','bb553c7e-d7cc-497f-8a62-5d5d21943218','0bbc2531-e217-436d-8b75-1d592aa226db','fafa8263-6895-478b-83ed-c53da45e438b','d19e2078-79ba-48c6-9d3e-36bd4a0d310a','f6d24223-86d3-48b9-8783-9faf443e0559','a831dafd-ebae-40d5-9687-07108aa988a6','5049bfd5-6e2d-418c-972d-696482ed2ff5','b5dee51e-8be9-4066-bdef-886cf4b8b04a','91b5ef17-e630-4030-8da5-d5e32389b7a8','7c3da91d-3f9b-4e67-93d8-b6a95b5cf1c0','33804555-52e9-4ee9-8edc-94d5d7a9e962','a718319a-6fd2-479f-b05d-6bc2c1b7c89d','07211857-6de3-4888-b7c6-95f5232fe211','1993f4f0-ba41-4b10-b048-79d3c991fd1b','16e95271-d21c-43ec-8347-8133688ee600','b0308831-00cd-403f-b107-7f8d188ed039','0ac72c07-d246-4a0d-9543-517d983eb2ef','69c2e280-2df2-42f8-9d94-b3c0ce6927fc','3485ec4d-2d6d-4401-bf6f-f0575c4bb507','cc74cd82-9e36-4f3f-a09b-8d89320b1f7d','d05d1cf8-0966-442a-abd7-bad5286dd13b','977d8944-63cb-497d-b4b6-e9a87f1dc696','30518b02-f748-40a7-b620-6b9ffc476e3c','0f2146b1-5b5b-457d-b890-ce817929ff23','ecb72b26-9f6a-4ef2-8825-a15c429755dc','23351deb-ddc9-430e-bef7-837954479eeb','b6026fdd-bce2-42b7-9fe0-ff664c57bf66','69042afa-84a2-453a-af37-ab8f3550224c','9602f1da-5d17-42ea-be17-ede167dfddf8','849069db-666d-4ef4-b879-1ac4f9501201','cced3dd7-f158-489d-84d8-c7623f919555','7202f35a-1db4-42a4-8510-15bdccd7cf9d','9709fff7-4391-4ded-922a-356110e53527','4cd04f4e-223d-4810-87c7-8837a3895c14','e0d069a7-2ea6-4322-8a45-f722302aacee','c7d1388b-a880-4774-992f-ba2b3c1d2a86','81f6b51e-f9a5-406f-a1c1-6274f31facb7','89ece46a-60e0-496b-b871-e410172c9198','0229e266-be29-4dfc-aeb9-987e4f688755','e5e359bf-fe14-45e0-b88f-6fc7ef53cfbc','1b2cba52-396e-4d56-81a8-13c23ec1c1ae','4a12b7c9-5ab5-49e9-b837-faf7c61d1e25','ea3f06db-7f4a-4dfe-b214-33b99cce5181','eed22212-d1a4-466e-a433-7204b845b54e','a165999d-abc9-4547-856a-22f0aa5252d7','1e5c5f49-a2fd-4262-94ae-4e99e94e77d4','1b896bfd-877e-403f-ae54-ac356fd1bc88','a9248c54-37af-49a3-84b6-cb64634c76b1','9d4df4ae-a639-4e02-81dc-c3a49341267c','117a749c-fb01-4630-8d59-87c426d507e9','1a08a8fe-9cff-4c3e-813e-22fbc4d85606','7495321b-62d9-48b3-9e8a-9f5dba610af5','c01f6e0a-82d8-41e0-af45-caa89da0a6d5','3495d65b-21a5-49d3-81fa-6276dc4bc52d','1fa504b1-3e04-47ce-adee-3103e6369718','1cfd5bd5-c5f7-47ac-8e39-c6b5eee56ea0','b9c094c8-6460-4135-9957-4c7e2933551e','4f19d8cf-8751-410d-9e4a-7bd3763f9d09','9208b156-69f7-4027-857c-eda5f6c2b867','ade7fbc6-6251-4cdb-849a-27138988f6e3','6522e043-c246-4ea9-8672-76c9202642d4','f3ffe969-cfec-464a-9e41-985ae1320d3d','32baadfa-5171-4a34-92a6-41f2f9638f1e','a5fb73f4-c373-4a54-b2e9-73e7a6fb7e02','2e24d91b-43e1-4e48-8022-d2a21c866fbb','078c02a6-89b9-474c-8c26-754acfb0be4b','8369ed8a-798d-431f-95e4-6df2e931b125','747cf0fa-9a57-40b7-8d03-0a1c57ebbabe','98557a68-dbd9-4c13-96ce-74508481267b','17d6676a-0aa7-49d8-9773-cd2e6e1bfedb','f221bb5b-819a-4ba6-9c9a-cb56a4ea28ae','55511ca7-6673-477c-9ab7-f4b686f531b2','48b4bad2-a277-4b9b-aee8-bef8d4b1caa3','45dd3801-df1d-4b2c-b53f-f14c187fd045','84e33c90-62bb-44cf-ad43-0a1d7f27b5a4','8d038347-032e-47b9-b3ae-8c837a4a5cf5','e74c6e44-7940-4632-8e03-e77657c65b62','d5957292-3d1d-48a7-9755-72cb54a3c3b5','0ae469a9-7edb-40a1-95e9-bbfde2132c69','028e61cb-68c4-4c54-95a6-5869555fe5ff','f24c1510-e7b7-4126-b32e-224965ac4af8','8f079d9b-6625-4622-a827-136986f993a7','55da7f90-6369-4317-a04d-a3785d83c239','8928c255-4521-42f9-9d64-2052e9d68098','9e57981b-48ff-4986-a63e-728985379534','14f4fdb0-db07-4f9c-af00-9a18d42a5b28','4a94d6a5-e8f7-41e8-8ce0-146ec1e31df4','5cc3dc99-5190-4ff2-8f0d-69ae7f2626f3','a17034a9-f59f-4b8a-a209-910109e48d3f','269678c1-c27a-4ae0-89d1-58810b63854e','571c0dbb-e0fc-4c72-a5a8-7dde02ee6895','1f8f89f6-8e32-4854-a23d-7e7f08631e3e','76b7be39-9ce9-4c5c-a3cc-05eac1367581','b8aab2b4-9a8a-43d5-a138-ded8ec3a3d9c','615819d3-5088-46a9-9e80-bd30fbf0871e','9749abca-7a33-4bbe-a9ba-8ee3c0b19a08','beff5561-8ed1-476d-8f92-f2c182ae294d','bfdc9c63-8764-4f30-adc8-58e81db43062','8e40be52-1bcb-47af-8ef6-d358c552dfd4','f8bb3c7d-52da-4c2e-b562-a38d121a3b2b','0f8c05a3-da39-4495-b499-c657ec511fc1','01a4c9c2-4835-43e6-b9fa-f117fb522b52','f81a79a6-85a4-44fd-a095-a05da3ecb8bc','5891e754-0f5c-4d20-a3a0-476590424e3a','570d13a1-56cb-483e-9e62-057e3d68a1d4','563c838e-55d3-42e2-ba30-cda55aa62f87','c67702d5-72a3-4eb9-b538-2c9f55f6070f','c35e01e0-e016-4b99-bba6-7d7da9d5bc53','2b4eef1d-391b-4bb5-a3e1-9c0bed126ed4','da56b081-ddba-42b2-9dd5-a96a9c7d5932','0ed7ddfc-1ac2-4e15-97c0-afec15e4990f','a53ba9ec-b05b-4d4f-adfb-29f16b55d988','fb01613b-d5b7-4bd2-b9c4-1b76bf679689','05ba0bba-dbee-4175-8894-2968eba273ce','9809d2f4-106d-401b-837d-21c79554fe09','b0b31435-0548-43e4-b13c-237f0f2fe4d9','a7d907ed-f971-418b-bdf1-b68550d780af','6a859c8c-01e2-4437-ae3a-4b046a7a2d02','57d8d81b-f06b-4095-80ee-a0a7e4b33b53','00294092-1580-4ad4-90b9-470936937bf1','106477d6-cdf6-4cc2-bd85-3925f51cdbc8','e323b575-2709-4f75-9c91-ca041c28dfad','83e4682f-03cc-4e9f-8819-650eff9610b5','2df706a8-6d95-4d4d-9438-dd4f8a4ebde0','c8595e13-6119-476b-bab4-ff4178ff9af3','cfca5596-3f65-43ef-91c9-eaa7f97e2827','bcc01ca2-87db-4900-b43a-bf05059f792b','9bd097aa-6c60-4ce9-9c76-ae7f43325f3b','f473603f-402a-4dd7-a4c4-5d6b429e049e','365bee5e-761b-46a3-a15b-ce3eaae05702','30173291-7be1-4eae-9d7d-54c970a08b9a','51a79717-64ff-4c6c-bf29-dabf4906ab91','a953761a-e07f-48ff-8fe6-b4712b8833a4','cae181cb-392c-4bce-9326-026e5fc202ee','51faf103-eaca-42c9-bb75-7f4408ab2397','d1156f43-8856-45f4-8a38-b75113cdfbe3','b0cebbe9-3fbf-4ba5-8eb1-a72715647190','ff0da62f-053b-414f-8d64-6be9795909b9','2ec50f23-1ff8-4785-80de-822ac2a96c4f','d1198b32-50b5-48f9-876a-5171d1868d06','76da5ba4-dd5a-4872-95d3-b67a30726770','f29cdca2-f5c3-4487-b425-5db5fde5d208','53fb7eef-18bd-4ec1-89ad-a25a9224d850','a60ad0fb-cc58-4de2-848d-4c9ac610593e','9a3f44f8-2a6c-4dd0-b6e2-410585d4a1f1','3ea1b9da-3ff3-4a75-bf6a-2499a8e272b2','5712d416-1adf-4151-8c7f-569c01bc1085','74b6d754-5c96-4770-a709-af96ddaa1fe8','a9d845ea-e055-4219-bdac-6de02874632a','a14dc6c2-3985-48a8-b4af-1bf1c5b860ac','79e09a3c-15ea-4ccc-8344-8906e0ca4352','819c0c77-788e-49a4-9929-07f3298cf1fd','b8edd932-4963-4d1f-9a6b-f5018670e450','36660a46-5c01-4d84-b252-a34cef8cfec5','0216e08b-5949-4781-bcf3-960a728319cd','845a6550-a5fc-4a5b-bbaf-01e5e88642ff','f2024c46-8e19-4cf5-9a74-0d0fffb60118','5e1589bc-bfd5-4c7d-9954-1be9a6be5350','16de771f-a719-4cfe-bc8a-648e7d3c6072','194ff108-7abc-46f4-af58-f1f19a61bec3','6e61fc3f-a38e-429c-ae9e-095b9fa57757','30660f78-ad83-4e59-90b9-681966614710','bd7cc0c2-b50c-41a5-bd3d-1c8a9aa871d1','5ea474f4-9b71-463e-b3af-ce0555298b85','7ddf9a6a-e775-4a3e-90f9-189c04650000','d099b792-047b-49d1-a3f4-0fa40c6f25df','81b47dad-9e2b-416c-bbe6-86c761a9eea9','f87c74a1-a582-40bd-8306-e525d517a043','24f9394b-af31-4f7c-9467-0ef322761de5','2c16a803-54da-441a-8f78-4a789b13b1ea','17a8df2d-69c2-40d4-87a5-5f6079a3ecb9','f4b8259e-af0a-4e8b-899f-4d5b583fb13f','60d66bf5-0335-4b49-9133-1129717fe617','8548ae08-10a1-4c29-a72c-fed1a8764365','3c483a95-03e0-482f-a2f1-82c461630178','909f0a8d-6a8a-4c0e-a055-129b10193280','84fa3351-d532-4de1-a334-e281b39c2841','9e1621a7-c113-480b-b725-5b146b086e09','8b90e817-3438-4710-91d6-8482b6736cff','b419c43d-0cb2-4100-9435-ac6de0f8ba34','38d90e30-e7a8-46d4-b02d-68d828ef8b6a','70e874b3-4201-4527-8651-67c86fc3bc41','bed057f0-b42e-421d-8f99-b185756ff2d2','28b30691-8e04-4104-b979-245dfc6aa04f','714b26d4-49c4-493c-b756-365dd8a12f31','6922b2d2-54d6-4629-84d5-4e1fbd84b6f0','a4fbbf36-9c42-4ebc-b9fc-a0bad4f0f217','6c93f079-c1a4-454e-b1cb-418cdd4d691a','e319467a-7f02-4d43-97b4-52027a83e143','3979b232-ef3d-4699-9a64-ec74bd86edc7','b13581d8-1d93-448c-a38e-c9c0acdca0dd','4d41e94e-87bc-4533-bea5-637b8d123bc7','3444ae07-7847-4fc1-a8ff-4fb27320ab13','1f1d69d7-6589-4ede-8026-9b8c111dbdeb','5e433606-bac4-4595-8bd9-ca3e08a8f0c0','52671e65-a491-4479-af3c-f93eb06e3511','ced860e4-ef2b-4f6e-83b0-31da788ca4dd','b4080055-ebcd-458c-939a-21f089460024','9c80a8ac-5804-4494-8678-55d7372dadb4','6480a641-df3c-4740-85fb-2d4b34bb99a9','86e70580-1756-4005-be44-55b946c20333','e6b89555-23cb-4342-a800-213fc2744cfc','a472d2c1-b21e-4535-9c05-1bbef15bc6b1','6031bf72-07fc-4b78-ac6e-1291739f4f41','1bbdce68-6870-483b-bc6c-163e82ec3287','643fc7f9-aad4-4d6b-b462-e32eea424a28','07a21088-f00f-4f91-9546-a866fccc26a6','d7a9d160-2d77-464e-866b-b9a14be76601','8bef5d53-5046-4538-af55-2b25ee04da12','6629a402-8d82-4976-b822-e1b516ad26cb','2649477a-4694-4ef4-a665-93f39b0042df','6336d879-a287-4d79-a946-fd07f7f205d6','fcef38fb-ff85-4a93-9651-1b8905fe2d39','dcc0ec80-f56b-411c-9ea5-ee51635a12c8','ed3fa485-9892-4a3c-8025-65214e4cebb4','9d9cbde6-5556-4f33-a0f1-e90278278fac','95e00d8d-fe00-4af7-88bb-7cbd0cd0c60c','3465c6ae-8830-4e0b-9fbc-d68ac77a00ed','fcdc0500-24b4-40b3-b255-602476d1b319','d02b87b2-79ce-4922-96a8-1a22296d1ced','7988af46-6a98-4d24-99dc-03cae53064ee','371e43ec-b85a-4bd5-8464-6c3d8010ed7f','420b1416-754e-4004-88fa-420807fd199e','965dec4a-f9f4-476e-8449-7b2945e6101f','5cf90d45-ff3e-46b4-a147-a393b625e4ef','6be2ffa2-c8b5-4cfd-a566-0b0e0f4448bf','55de3a3a-01a7-40bb-832e-5830e3afa022','b00a3948-fa26-4ad3-8fef-a0fcafa8aa3f','abf80025-1052-415e-b18d-ab1a93be454c','7b6e88a1-6632-4c1c-8071-a761ebb4fa64','616ff0e7-a852-4444-8a48-914ee2274a08','420517e9-b44f-419d-af65-94ed3c67385b','d429ed3a-521d-49b2-b73b-282c1f52fd6c','7b3a72bb-33f8-491b-a94b-2679f46bb9db','cb2fac37-b8e2-4371-afb2-eb0365b2319b','12f878df-ed1b-41a5-a633-a4ca1d2eabc7','c0f25702-93f3-43ec-a6c8-e7c3dcb319a0','0ad9b005-7c8d-494a-9b26-fc77212974b4','867d38ba-c5f3-494f-bb98-9c5e20e253c3','0d8b13fd-9437-4037-8f16-31b20b543828','9ead8884-1706-485c-8f73-9d57e3d1dcc4','5f6cbd6e-12cb-4278-93f9-9778ad135d70','3e5e5e88-7c8e-4a3a-9782-b2875db409b9','c511275f-0f8b-46bf-a155-b7580a3684ef','d25322b5-810c-415a-aeb0-ae0e5ac2a7d8','287e459b-0502-4a48-8b7d-43d8f7feddeb','9792d383-8296-487c-aff7-5fc63a7fd4ea','1e6e3176-4248-44a3-9b8f-0e3dcf9f0b76','8a3618b5-d0fc-424a-9fe1-605741d86f08','48c8f831-0f03-406b-bd24-21db3e3db6f8','7e12fddb-e34a-4b40-9367-970fc41da14c','a4199a73-f6bf-445a-9ec0-e87e521f4d56','aa58e9d7-d85a-415c-9b93-f8e6deda2c31','637a338c-d2d3-49e8-9919-abacc67ddbf9','493c932f-2252-4180-98b3-dce9b8c7cf57','abfa366d-fb79-420c-accc-55c0767f84a4','90b44fb4-b8a9-425d-8e81-e8a1b10ad453','01e5c554-1457-4c71-911e-a400c31126bb','33c1f73f-133f-4d14-b00d-1919648ecf4e','640cb757-e87f-410e-803c-a5a50d4be1ff','25c10d08-7659-4e4c-89b2-f6ed1c96ac9d','3a1c7f42-00e9-415b-8fb9-20734efdf801','a45893cc-0013-4653-bf3f-0c0fb921ce73','67699311-fa5a-4420-a710-5c00d87840e4','cf2ab16b-dcce-4e17-98f0-e41070f3d6b9','bd44a115-7d33-4f6e-86e8-6f5de7b9e9d9','6d29fe65-0c0d-4b8b-b14a-95974e10a66d','b6c253e0-3fc0-41ad-9c5e-c789f7940527','8f615a61-3b84-491a-aba1-d0e92f9ee507','6d2b3eb4-22ce-4d9b-a7d5-c497a42e00fb','3e4f0a09-755a-45c5-8f2f-85ba4995e3c5','945ad68a-d9ff-468b-a9f8-6cf10568c2ee','2cb1ec91-cd23-4512-a0e8-10f565dd20a8','dcc4a471-abf9-4768-8fc5-2693447e4ee4','d8835557-4b72-482c-98a5-3b93e0e2dda8','c2b9c7b5-2a2d-4c4d-8114-4cc3e2450260','85632127-aa55-416a-89fd-55ae10f89fbd','fad5756c-27de-4999-823d-8f7b5e7914b8','f48b668b-a221-4bf6-9137-1ae80ace4ce7','005f346c-1718-4311-9b2d-66d4a6e2b702','fe08e69e-8ec4-4415-b19c-3a3251b1d0a8','c2130073-e316-4f93-9e82-2ea3ace4c7c5','6315a82d-72a4-4444-bfd2-add4b32434f0','e3ca91c3-3363-464f-b5ec-144eebc6e595','11deaa8f-5abc-4d0c-bb5b-debf52c4605d','57370956-f222-49ca-9524-457408a19750','6ffadd7e-8aeb-497e-a3f7-065b64b99b83','28ff7e20-5454-4bf8-8080-a4a4c0d3552b','86c98311-5510-48ed-9aa8-425597b9143b','82054220-bf27-4d2a-bf75-f132e3d80545','ea979812-f394-4330-8f11-7402c360e817','a9a949d0-97ee-4b68-a466-ae81fd3fe55b','6c3ca76e-7b9c-4813-b9f3-cf7ea93df5b7','c72febac-b147-40ea-aa3e-e915bd391195','2cbcb551-19b2-4639-bc93-8e1768331185','e5e9fddf-4a27-4d4e-8e2e-2cc2e6c384d4','d336aec6-d888-48d4-904c-a99131f009dd','d7b72a2f-f23e-4b70-94b9-18a8577223df','ca7d32bc-5e4f-4493-b05f-0b6b6b3f8105','3b340d18-fde6-4c6a-9872-65573e87bbba','5b3612ac-11e8-4f86-b336-9e7d926bde8c','1e1a7b71-1378-40ca-be8a-569e208e4657','408a3290-6934-464f-bacf-81ef991427d4','00cf395c-b4ee-42ff-a2a9-1eb702743f10','24ba00d0-097c-40f9-89c8-13122d0af313','ae045d13-64ce-4f7d-9ef1-4aa0376a2825','9ea60062-d827-4074-9e97-b1ab21805aca','9895afce-bffe-4015-8a6b-bdd0b21599ed','168c8748-5800-4474-b095-6d8e8f31f7e3','f337bf43-0a03-4a35-a236-aa56b6b9dfec','f629f8b5-3bcc-413a-8d1e-bcb9375d15bc','fa8ba47d-d63d-4600-9ca2-dd5777e46b28','181f69f7-c6ef-4230-a105-3dd0e67e2d3e','793f22cb-50d1-4fab-8b08-b22baad128e5','0df73f63-c91f-429c-a616-79e2fe5e410c','4915b797-dae3-473c-84e7-d7fd57ad1bf5','ab279e32-a7ed-43fd-a7f4-69ad24801938','4ca0bf4e-12ee-40c0-9779-8e20e464d93e','38515013-8b25-476c-9cf3-458ea5ad113b','b32f8f5d-e710-4c62-9d06-0b6360fc391b','8bcd436d-50bc-43c3-af8d-7ad3ca956b71','b4575a64-bfc0-4ab8-a98e-f532a768c0b9','3c4bbc70-eeb6-4e29-8753-ed164cbd2255','ad347714-230f-4373-8406-31fd5b4f0823','0a3e8bc0-ca3a-4b13-9e9c-63c7b85ec023','7551c7af-01be-49f9-9d4f-6e39e30dd191','3002310a-14dd-46ba-ad3b-d5afc128139d','d334b782-9bf0-4978-bd1c-131862065e08','34577924-e2d7-4c5e-adee-84083aa8b1e7','842c06e7-f352-4689-bc35-401273d6bf2c','a11223d8-6a23-4805-a908-48c1be495333','198c51b7-3f24-400f-8630-9c89cd19a024','01f0bc15-4974-4048-ab6b-f90d9d41140e','75c6729f-bddd-4e83-910f-a40c9175f3b3','c730c582-f459-406e-b6aa-724824ece9f5','53b8d73c-7402-49da-bb0a-7cb3071e2330','c327220c-28b5-445e-bf3e-3a86d7c44bf8','1295c4fb-1fba-48cb-947e-3efdb888c425','2b589c00-b43b-4d3d-a534-a980cb9c5540','f76f6ce9-4039-46a8-880d-4e468af6e7ad','a0e4c38d-9a23-4ea5-a291-f7cf89f13520','69fb2a23-544d-4dd1-adcd-dd6857b920f6','554055af-f361-41c0-98c6-c02fc7b12a00','e995ae8f-df29-4fc2-8061-952e24e8b3cc','346a954f-92be-4162-a3d8-4cd8ef95638c','0e6a2595-7919-4ae1-b969-dbf49bd2005c','f34191ca-ddf0-45fb-b271-f8ad260b9920','9f035d57-f6b1-44cc-8cb5-8760d21c7f80','959cd4e1-c805-47b6-8fbd-6028930f1bc1','690171e9-42f9-4a11-a022-cfa6dafc9b12','939b0849-6328-4242-9831-8d695fd2747d','15fbc9c8-7267-437a-ba51-9827be8f974a','f91e3ee3-d7d0-4539-b096-fdb15ee7b9fb','ce16181a-1044-4590-8406-85d317a7873f','e42a9b6a-e8f6-480c-b607-5522601018b0','91876895-edf5-4f10-840a-16541b888786','ca2ce98a-c7e5-49a3-b20f-4b525fa8a90b','93f75584-6407-4091-9ea3-f5cd32f3dfe9','02da6d29-8557-4f36-82c3-2b157cdf09ee','f8f413fc-a673-4b6a-a8d5-0ce1f16fb604','0bb2a481-e8a8-4cb8-a69f-c5ce718529f5','9c24ff22-d37f-4eda-b864-a95faf21f29a','1c6893b9-d2e7-4677-ad39-7674ec5a69ef','b74562ff-0933-48c1-bb66-6df01c136024','8a149997-c5a3-4926-9852-82a84b0a862f','51726d46-7d5b-44f9-8555-ec8dd06c68c4','b0a7e81c-d3a0-488f-83ae-046cc185c174','3197d9d0-93a5-44ca-9218-fc815fdb94c0','a56e24a8-7307-406b-aebc-18abdad09985','4f531313-d013-4e52-be40-1c7a4e7f03ce','aee1ea84-acac-4462-a2ec-a31448e0d9ea','133e0d0b-8281-468f-8eb6-b4d0b9a5d0f1','0d133182-7a7c-47ed-b0db-d22cc29f6b40','e4a1fd8f-4130-42db-a375-e47b0c5c8fc1','89a8ea4f-5425-46d7-b79b-9852455fe102','feae0ff8-5b24-42fd-ab9e-f28caccf0b42','4cf17383-a0e0-4c14-a1cc-601d9c022f79','ca4c7683-2eaf-431c-89ae-94251257663a','10d0fcbd-3be6-4608-a551-de3e7fb5d38f','997439e2-cb56-44e4-a317-3d41f1098967','7e8382d5-22f6-441d-bed9-b6a94abc37e3','7ec324d1-6bf8-461d-a6d9-c9a6c07d84f5','135217a0-b7f6-4063-8a63-1be2bb08817a','124f3d32-ced3-4cb3-80de-437a59e177ad','c4a93f13-a893-423b-92f4-f0242a3ee623','e85ea2d5-6e98-4263-a6ec-edfef039cb02','2da116ba-1d2e-4b7d-8afa-1158ce08ea47','349e3f9d-9db3-4240-a855-5457cf74f01e','d123d874-5d7c-4514-8a27-bfc4852e46cd','522c792d-9f17-414e-a389-93281b3bf187','f74b3e2e-8b59-4928-b7b3-9288e1cb6c7e','dda3c18f-9888-4341-8a01-0003f5877133','982f5210-2ae2-4923-b090-1f34d15dc6b5','53df6b4f-0611-46db-ab2e-c070fe517853','28f84563-5946-42ed-b942-0a4f7539417b','04768c0c-358d-4bcf-aed6-41be2b3728ca','43674891-39f5-4a91-8cda-a38419301a1a','4e767f50-ab43-4016-b53e-b19daef34a94','0b7948e5-6e6d-4b66-b270-d9d65a88f43a','09c5b933-ad21-4c23-bd6e-e66dbe9b8627','431599fc-c67b-428a-b930-dcc6c77ea04f','2de3db0c-69a6-406f-ad9b-6b2993821ae0','7b39b394-deaa-44d7-948c-99b5063ef1aa','635c509f-9036-4d84-b30e-e75bb3f17dce','07706f67-6ec1-43cf-bf2b-e2c86f34bb9e','f114ddfa-2137-41eb-b89b-f8450059a2ed','3c3af090-567d-4eba-9eac-49c0042b6322','8272c51d-7b62-45e5-8eed-c2af688e5a75','a069125c-da51-487f-8ca1-71bd89ac6fd3','4b5fd583-0501-4ac3-8abc-ba13bd060f8d','b7366796-7b7b-44ed-bf6f-4fb532908fc9','3290bf55-c793-430b-8192-2f28c6465caf','333848c6-f082-4f60-bea5-898e160170c9','22b324e9-6665-43e5-876e-368be8aa66f7','3189fbc3-b2f5-4e90-89af-85e56046c47e','4d3ec812-f38a-4189-a529-201acdfffa2a','c15ad1f0-7242-4c25-9c5a-cbf7f3a536e9','bbd14ca4-9f51-42aa-aad6-e340a2aee1d8','5ed0542f-bef8-41d2-817b-c0f76c125d6b','1f133d82-ab17-44be-85f4-0212b6d7bc7a','2f6f9d8f-7018-4c8c-8955-3b8ae713f6e7','7bfcde32-4d33-42af-b21d-bbfbe0d48286','6a7d576c-2a62-4e12-9135-a6b22384f9fd','94487c89-528f-4db5-abf9-674006ed58dc','87aa69c7-4d6e-4da5-835e-ed7802192569','92f32617-b322-4d87-8754-eb3bfbcd5a65','08616f8a-831e-40c0-aebc-bc032cd2927d','3801f6a5-ba98-4bb0-921a-efbb22a34fdb','215d4f6a-1b2f-4fd5-924f-e6fb9ef93548','4f106f2a-3037-410a-ac5c-8b6611d01b46','f22e1680-a57e-49c6-8b16-246db4f5cfb6','736c92c7-2e3c-4dd9-a7d5-7ab15b1a6842','22065f6a-bd1e-4ab9-a469-e8e57e6e74b3','41c3b76b-3cde-41d3-9f02-a5a2ba0d3ffc','199a8280-9260-4026-9b2c-a8322a9f4986','349f0ede-84ad-41c3-af1b-5bc37ffec9f9','77e95c79-eb95-4f10-b71c-2df3fdaaa144','8360fde6-a5b8-44c6-93ff-3657ce48f9df','3bad1a4b-de10-4e90-9518-5b2d8a93c3dd','48afdec3-11d5-4f4d-8501-5d625f4fed69','1d9ecb1e-7b37-4da8-a3a3-37d8e48ef57a','20039516-de1f-42ec-bd12-3693f88efaff','553b976a-7d3f-4fed-9314-fc275941b95f','5a845230-df8d-4760-8c1d-0e8d907fdac6','9a21ea2d-3c66-4382-bcbe-89e13072e72d','9cb4567a-3be9-4e45-969c-641559ed0b75','a99eec36-a2d8-44b4-a6da-68ea5627e501','91834c1e-f594-4e70-8c9e-37d0e3978e9b','37d14a85-14f1-4463-9270-f7015941c0fd','1bdaa64c-8a30-49d2-bab1-14514c65eabf','9932c124-4b71-4e99-990b-a8e0b4c7f208','d662c079-2941-4cb3-a26f-218f7e624326','ced5de08-43b8-488c-85a6-a47d430d7248','d8f4c26a-0c3f-44b5-80fc-a1685d876012','c9732d41-8309-40f4-b92e-8dac9c893931','24347b2f-bc95-4e3b-b82f-2a5db7c79e40','50ae73ca-e178-44ce-91e5-bb9ee89c20a8','ac3ddf6d-6028-43ab-a18e-3f06a1701f1b','e3398fbd-f079-4e56-b082-4e16361d7231','a024fa8e-2bf8-4257-910d-0b36d21e080c','497aa944-00fa-494b-9d24-edb26af38c4c','c98706da-5dff-4356-a2fe-fef4c60bdd4a','e6b548cd-8b1b-4717-96ec-fe9f33edadbc','411773c2-4e71-4985-b302-77513f5ccd57','dede4687-cf5a-4813-9d60-1d8ca154a238','6e63ac27-b8f8-4067-bf01-0a0a69a23251','6ca4a862-c9bb-4f9f-b2ad-8ca020ef9ee7','667852c5-2911-4e4a-b4b1-d933c01b7265','bc0a02c5-83ff-4976-8647-37f38048d440','50d3e4b6-b49c-4d5d-ba86-e8ba6284dea7','ddf9ba69-dd29-4ae9-9fb1-c797554b7d61','4ddc02df-894e-4fa9-ab47-f62d06d9b47e','5db0fded-0371-4b07-a962-3e5d36e1dbb1','17f1eb27-b62c-4dd9-9999-cc0269ffa184','fb092680-435b-488a-a72a-880caad45846','4f5061e6-3a96-4e8b-8064-461a03e3608c','4fd73c7f-450f-4a8a-95b2-2c4f822f28e7','f5ce3279-a9bc-4ff1-8f6a-700309ab89da','7b16eef4-fcc4-4c77-b6b7-c357ff32da76','f1413ae4-9cf7-4534-af54-752c67ea4b62','729bc0ff-784e-4741-99e2-97ef28277aa2','55929f34-f511-4679-bc21-8e73c0bb7793','680fdd93-ae70-4c50-a21b-a022615b74c1','b403e030-624c-4109-bf32-a14f57f0006a','a0ab3544-b0a3-4af3-881e-0a5d1caefda4','f85b52b0-d9ee-458e-8cfc-ec59be733c18','38e5b16f-9e47-414f-885b-43ceb06079a3','8ff1b207-9c56-4ea0-afda-bc52428e1783','809f1594-286a-4ef0-82e2-31776b1baadf','bd4f9ef7-788e-4c94-a4aa-b5be2c19ae0f','a310d4d8-144e-468d-a0c4-1e80ebed2b1e','b44782bb-4008-4633-8525-dfe4ea4ccbc5','f3e4a77a-2cf7-49df-95d6-223fc9675ca0','cf7b414a-740e-4436-b7d7-9a27d5fd69fb','e816d943-1825-403a-8cad-4c03dda65941','52218897-5ffb-4dc5-81cb-c912b039bf4c','dfad05c9-98da-491b-b80d-d3f33b5aca0f','2f8c1bc2-14fb-42ed-a4c9-ddddb54802f2','0fb1d5cf-b346-484c-98bd-d43a70af6a90','be55f426-b9bd-4eae-8884-471c1cb7bf73','fef0a83e-48d6-4fbb-a742-f31338c5b00c','dad2a3b1-c279-4c42-8009-536317d103f7','21474894-c733-4de2-a173-319320e7c3bb','73ff12a7-347c-403b-b183-f5d4ba6cf86d','d1266153-275e-4ba1-b25a-eb201741c73b','8d7bf06f-7285-4ca0-8cd1-9aa241b9bb87','357c067e-2041-48a3-9063-7b71c6704986','5482c115-fa4e-41ed-81b0-f6aa6e0d4339','1e44e297-f964-4edc-971a-01a44f698ae3','707f9120-a656-4fdc-bd05-f36805a084c0','a225b814-7e59-43e3-b3e7-e861d2f2a4ff','d75b03a5-4fed-46b7-b31a-4b636fcccb60','aee4a782-5fc7-454a-9697-c9acb326e046','4fedff28-bbd4-4aa7-a5f1-48d643c01984','6ea2d791-fcd6-484b-a882-ebed3dbe3b80','6d4d105d-b399-456a-b9d3-f515504a73ad','0a5ec3aa-659d-418e-bfef-37787940e55a','ec2b1b5e-b61c-4d98-afdf-126f8425fb73','2d211c73-a646-4145-be02-f8963882906b','39c7c6de-535d-48b3-8656-ac0d585dcbae','e58d2d7e-ada1-4d06-8ee8-f94be37c58e4','d655648b-0586-490d-9611-45bc79dfa033','526fa02e-3857-4bc0-a8ab-764b7f732956','a1340236-f971-4924-a09f-d84339967155','dde0a979-5fa8-4913-ab3a-a2dd10872e11','f51e07d0-e8b6-4b64-aeae-71e16ead5161','cc913aea-fa70-4927-806c-99587519cf02','bf2e536b-5a52-40f5-8cd0-754a69d1dd0d','5eaabaaa-3cdc-4b5c-8925-f1598eb0ee02','0271019b-0a28-4598-a6a9-912172107f7e','3c019653-f581-4e92-b2c5-4c8083c6ab3b','91a631d8-fabb-404a-92ba-f260781acdd2','2743f3fa-c833-4e7c-b044-79ab6c9759c7','83d48871-fd3a-4cea-9158-e9e1cf423503','99a4d51d-401d-4421-b962-3e39bf156c93','11e77b75-be29-4c2e-a93d-36d9f1a7df12','5523b4a7-340a-4f11-8f76-e3063d7d0555','3e499704-ec06-4892-8345-d935f5915da1','0b86b349-0679-4619-b41b-7bfd68ded72e','89dd70f1-a800-4562-af35-e19f38c6b6bb','538611d5-9118-48f4-b144-e9be55b4b7ed','5b0ca56e-a137-4932-986e-4d057d52f410','4dabd6f6-7e0d-4d23-9e14-5ec38376d053','0c998e83-2045-4f6c-a0e8-96f339244797','e14a7082-249a-44ff-953f-fc96ba05665f','c79cdb8f-09be-4d21-a400-b0208bd575f8','14d9fdc9-6c31-4313-b2d4-e7935c97e7d8','658f065e-ebcd-4c12-b78d-aa59942ac3b4','2607e40c-f695-4981-8059-9882e37794a5','fc1cffab-5c42-49b0-92e1-43c974774058','ab10a15d-030b-4a66-9b66-57d3832f8fb0','3ec68f34-7dd8-4e12-b71f-d5b42c689ac9','e9573acc-340c-472c-a9c8-6d8e666fd8b3','bb9ef764-e69f-4a7e-b3ea-41cc4672a1ca','2ad4c9e6-6e82-4115-8fac-0e30ef74ad39','baa741bf-bff9-4485-bd7c-0de35116edb1','65972019-a40e-47f3-a563-79612f8620d1','8937bafd-12f3-4a3e-89d3-cb5348958bb7','c69518df-c359-44a9-a7ca-d2dcf97f5d4d','cd7aaad5-f942-4854-ba1f-84ca6fac1793','bea5ce62-63ca-4fef-b0ff-1bba4ba68036','5a28af81-86e1-4aab-ad60-9c6491acc523','479693b9-d734-4a5e-864e-87dbc3cae4ad','a158bd90-22e4-4d48-93e0-6949618725af','e0107f2e-5ba9-4f1b-a173-084d892d1a90','ac0f2f31-4ada-4682-968c-2aa8f1ae9778','150a58d3-523e-4dcd-b1e5-b25952d522f6','c37edb56-6242-4fe4-98fc-522fd3e90c72','77c75c8c-adb0-458d-869a-07fe623b3f12','91bf91e6-f8f8-44a0-80c1-368554db0d00','82cbb875-ed90-4722-bab8-9a0b10afb5f7','0b61a06e-62c9-4ea7-b894-a2fbd9e0e7ca','b963ac90-997c-4a62-92ac-2547174d347c','b94b0189-2412-4cbf-a47a-deec0ff5af10','9276efc3-82fe-496c-9479-e5916f142328','2e161556-709a-4ceb-bd1a-cdd1f8cf7b58','655c19b0-bcfd-450e-8f7a-d4a47c34ae70','e3847d43-02de-4d4d-b549-5bcaa701e437','0afb4e5e-e09e-4f1b-8aa3-ca83e7ca1683','3619e1b7-d5dd-4121-bbe7-72c887f3fa8b','26827afb-9dfd-4c74-bda9-c60affd3862e','d3e17b3f-9b76-4dec-8f25-38f516e4f721','f7ba7149-c0ec-4285-9fe6-fb5bf57af4cf','917e27d7-12c2-4377-b941-bc7cacbfde9f','f55f85e6-af1b-42b5-832d-e8820b151b34','76a3b703-4c25-449a-93b8-2a5b0a16b946','90f78122-a68a-4238-b0d3-e446b44b6d17','c92da727-f928-40b5-8f83-875890263c44','1b73a63e-6bcf-4f77-bb0b-8dd42d91c708','97e0a45e-d1b3-4682-b855-3be345326713','1a62cc93-c3f4-4b0a-a092-063be0a6636f','b5632877-b782-4e43-95a6-e9f22e51eaf9','efaeebcd-bc7d-4985-8d9b-18fa7f533c26','cc8a6351-395f-40e7-9eec-36c69c284926','1ef2fd22-b13a-4bdb-a4b7-4dfd7ce857a1','f2588102-a4c5-4178-9c29-d9199bba025d','50703d87-bc62-4d90-861a-0973754c05e2','cf7d168e-4fae-49ff-8127-732e24d40835','c9d80905-7101-4465-91d3-cf52254218bc','cc0e6722-caa2-4409-b2c6-d2851ac237f2','f6cc2ed6-89ee-44eb-896a-38a3852fbc3b','255eeb05-a597-4f22-a468-bd8311a11af8','d0a97858-444e-4bd4-addb-49d010205f52','f8940ea2-ba39-4bc8-95df-de211e1d52ee','a715f62f-ec1e-4fca-912d-b105462562e3','d5badb55-889a-40c5-98af-9bc50e07ef92','5e8fd54a-5fad-413a-9c4c-1007a9878c24','e207277e-85e3-4688-ba82-0d2d230b640e','9214e95f-51c3-4216-aa0e-133e7caa688d','a2ce47d6-c9f5-4baf-bcaf-6f9017437033','8888dcce-351e-406e-945b-c40c2a2f92a5','1d2d3b6d-613a-4251-94a8-6b84e40d1e8a','2d34afa1-4745-4a5e-bf84-f47f5d9f5a53','4c6f244b-33b6-42f4-b8d8-7a703e5965ca','28c7b7a1-c2bb-4636-9e40-5d3a55db993b','39912429-fe44-40d6-9ec2-eb27d9936827','bd64808a-f83c-4033-88b5-5e358d561dca','16df5937-0f9e-4a5b-9c33-eb08051798ef','ea9c89f2-91d0-48b3-bef1-695fbba4454c','71488e99-9a0c-4c04-b568-6575aac0b32f','1585f05f-911a-4583-8307-8a3d5392ce6d','04b3d615-5a11-4021-8efc-0fad3709c497','a8f64eca-f5cb-4705-8384-094d75c96f25','882f1716-b135-4c86-a5e2-d9d9c5009cb4','b0e33aaf-e3d2-4331-8b06-4389ec3d1e50','cd1bbdea-89e5-4dcc-93e2-d4a8322273f9','a8b07477-8da5-421d-9b20-592651630db6','4b4b8058-66f3-429a-a75a-9692971a66e9','290fcab5-dbeb-447d-b965-2da35100ca98','f93d822d-39df-4531-9378-c2cf8141d10e','c86d1654-d1fe-4f52-a873-2ea76eae7fe0','459d9851-78b4-462c-8bf5-fa4f0a96304e','f92f8a8b-eecc-4a55-b9a5-a2fdb6f30cb6','e111e47a-5be1-4b44-b955-4027b5e9eeec','3d95f2fc-1ae1-4185-81e6-cf679e002b5c','f6feebb2-a7d1-43a8-94d9-7b2dd3de2d4b','d0247e5b-68e6-4a79-9eb9-19bd47789661','6f78beb9-8a5c-4567-bf8c-d7c33be35575','10a5eea9-d3f4-4fc6-9016-8be461d4cc62','74245b3a-ec18-444e-88ac-e7c4ac567afc','8a57ed90-5b5e-4073-a768-0017d8f626bb','73010817-5d2a-43b8-bc9e-4993c4700edc','ce6875dc-ad14-4822-8653-887a29ce1725','a528d032-f438-4a88-97ff-5aa0202c127b','510d0c42-0d4d-404f-a57f-c8568bc39643','4ffadbdf-c012-4922-9df5-2fb980bd3ad0','452a06b7-6da0-4c24-b394-cd634b914222','57b560c5-f5f3-42bc-9743-7d2a3dc9b8ed','de8ad26a-b9af-4c96-9880-d76a6d9ba68f','0148838f-fbe2-4f00-a23e-36d8ce6aa24a','1efe70aa-28d2-4398-85e6-552f184e14e7','eaee78f3-47de-4732-a598-f54cb4f31e2d','ebe430c4-0ec1-4280-85e1-ef04ab0e2675','1e538ffb-2065-4e9f-9a29-9267686a79ef','d33988c3-76ec-4e26-aa29-310a84d42ef9','e8fb0ca1-cbd8-4c61-9693-ac93765733c9','0649a419-74c1-4f36-9a8a-c7f552cb8d27','377541b2-8080-43a2-b19e-b06c0009b5d3','75f8df34-62c7-4556-b145-f696f037aa07','5357909d-96d0-44ef-9498-502ae0a9fea6','03349838-59db-4a27-ac85-9d8a9e1b382c','17b78885-ae5e-4171-8a22-2c59a65b31d7','b4b23945-b03d-40e7-bfe2-b8f2b6fe1d0a','6924a595-0be6-4934-9fb6-48be3174b779','ccdfc77c-8b56-4707-a443-6e5952f85f1b','ae772dc0-b1cb-42be-a57f-1bf6c7242d0a','be79205c-afc8-460d-9985-202f7f689ec1','8eb455bc-f282-4eb6-b8d5-31c318dccb58','3118c0a4-6887-4800-855b-6d46efd8389b','5ddf898b-b2c6-4781-b34e-65423ba771bc','dca719a3-03eb-4e78-88b7-8355dd1bb3c7','30dced64-8997-4b73-9f29-37023cbee0a4','29627a61-ec76-40c0-bac7-5f82647f5adf','18fd3584-bbd9-4353-9616-1aa8e22f24e8','d4544258-c8e5-4db8-9ae1-6778c85f1706','10513f05-be59-4f58-807b-809a5162b763','e7d88476-a1bd-456d-bd42-b0fff8b5bcba','85109dab-5f6d-4009-9ac8-95dbd28ce6cb','93ee7b57-98f1-4486-8cb6-3b6dbf1185ec','55dacc00-6dd7-4568-8d5b-f7b8fc4f4add','64a8f3d7-3679-45d4-9416-2d67668c3a66','f619c67d-dcf2-4a42-9999-a240c62a11e7','8b3a995d-c8ca-4544-95d2-80b3d30363ca','ff9c8048-4fd5-4743-a4c9-8e898377b0d7','08624137-1a5d-4a7f-932c-cf127b6e0215','1d07244c-00cc-4ff7-8a78-111a88e45321','09b85d65-ddcd-4b22-bb57-33336e978341','a6f2fdef-f4e3-48ea-86e1-19a6c82538a0','1f654c6e-117e-4f3d-a930-c51b19c32279','41603660-861c-4cda-a446-d1def497c9ec','4c835cda-8d97-41b9-ae14-b0a0a68f4174','7a002787-626d-49c3-be3d-1dc224373fd3','04528fb4-5a23-4280-90c0-9b0f21235842','826fb8b7-c289-4491-9920-89386578cdc7','c289c6ea-2254-458d-8330-ac1ddaf86ead','feb91921-3626-4498-93cd-11ae3712f494','8d319a97-7a14-4362-b534-4d32cc8b6d74','c6dd3356-8682-4529-84e6-c9cc43aa1d86','e7eebcb4-f157-4118-b997-e6f2ecc2c596','57872ead-3ba8-4d9a-a6c6-124f7831f17f','f835d9db-e5ab-4b61-8d7f-3feb78946e14','212b7cd1-7544-4e4d-95c0-7a51e6cd04ba','8baa8eea-fe3c-44c5-9b84-2cc4840aedf3','ede633c1-6bcc-4876-bb64-e06e0e49c7d8','129a08ba-1351-4263-8643-59d0ef781c0a','32e2f5af-0da4-4f40-8f15-446b1ceb419c','44f0f7a5-f93e-4698-9e8b-ddf7716f6c1e','db5a95ba-d868-4ee4-9a16-ce6eb527a3a4','1ee0bef6-754e-474f-97ad-4c71cf1912d4','9329c1f0-50ec-4985-be5d-d88f7cbbb319','ea5d1740-d199-4074-a238-b33810c8c903','ca491864-4455-469d-83a7-cfb4f6e105fe','eeaa758f-f82d-4260-a071-d157a8ff0fea','3142dbf1-37ff-449f-b440-af1906bacad9','8cbeb7e9-70d1-422a-83a5-e2b26ae6e875','f0fdb151-d4e2-4491-9b5e-a4516a74200c','ed77718a-0da6-4983-9267-d7b8f9fa55d3','fea93715-2b52-40d0-83c4-0002c96416f5','9cdc683c-e943-4b37-94fb-f465c089d5e8','3000dfd6-6bec-441f-8719-172b05f3591f','743ec20f-e919-4b4b-aa47-7f513355cc87','f637c375-6e05-4235-9533-63f597c5abd5','b3f53df8-9fe9-4748-833c-b198ff79f193','93e661b8-d898-4552-84cc-a8cd7e1f2680','ac40dac9-bc5a-4f5d-85df-916a069bcd81','70be16be-7416-4d52-807c-ed3da4be8ccb','82f532df-d7b3-42af-98ca-b0706fa93cc7','505df7a7-f743-4a16-96dc-6d689b8ef9ed','ee5189a9-e445-4c20-b6f2-1ada8068e717','5d98b52c-9ba3-474e-809f-bd593b138618','e3fe62ed-ead8-4060-8390-f63e73ca303e','5b03610f-0e94-476d-90b5-254faebeea50','ace5c7cf-de57-4616-ad35-48af54b8e957','2ec4c51e-f6fb-4255-9cff-f3777f62253a','3ab7eb08-4083-47f2-8c57-83829eb49cd8','f4188f30-c21e-44e7-8acc-e97d3af7acaf','c15d8981-a7ab-49e2-a74c-08840f9db380','8a4609e2-66c9-49e9-8614-30ec61d62baf','e764e74e-fe3e-4ef8-b20c-05e2a2608048','c4220f64-16a1-4fd9-a8c8-cf9e5edd8371','82e99314-fa6a-4ed2-8974-f2c719754b61','b36c7649-14bb-46c1-a996-056e3a9070b5','3f6d869c-d904-4320-a2a0-1047f95e450e','705b7f3b-7202-48da-8096-c140db7d7797','276fff29-5407-4a9f-8463-fd955090ceef','896a638f-ab7e-48a3-83b9-176e6d7a1fc4','aa4fbcff-7a19-4f81-815e-d9ea738dd19d','d2117fdf-ab71-45fb-9e52-92b4b6e52584','234b9bff-22d4-4ed9-a538-de133deb2a1e','54bdde5a-e0dc-46a1-9f9c-f6cbf5e07470','065b57be-46c1-4c17-8261-6568d291db09','ee05e202-b8e7-4184-8692-d2b90e7b0c04','0e6e839e-6ff8-4e16-bad9-1bab4640ba02','86d210cf-b96c-4d00-880d-3ffadcd60ddf','d8e452d9-ea3b-4406-9520-d14b7768e93a','9aa341ca-22bc-408e-be63-b15bbc1bdc0f','0dff7f1b-62ac-43f2-9295-a0a832e703e1','da988b4e-ea0d-486c-a692-d65c4a71ac57','0013aaf5-b458-4c55-a8c9-b6115c42d697','124ef4a1-16eb-482c-ab48-601c71a5f965','89a545e0-8daf-472f-ad50-8bc64536fdab','34c8ea65-3e8f-4824-bb47-e7fcabb526a5','37d43019-9d4b-4590-bd52-b18bd5c34c64','3c05d04b-a47e-4511-88a9-7d62ecabc407','121de1c6-2b05-4a9d-a0e2-6de44286f0b3','42fe2077-99ea-40d2-9418-b56e3454334c','ca5d30f6-2c19-4a23-8cee-53082a1b2c6a','a7e30782-6800-40e7-b141-4bd2302ec041','449b44ba-94ee-40d3-9b11-57dc97550a66','fa4bcfe4-c686-4b72-9f29-66789c89b976','a718f380-acca-4af4-a838-566f19952cc4','8e14b302-7a45-4292-a109-a7bbf3dd3e0d','f7d9d72e-cb30-4127-98af-da78d7203fa4','ba966648-4782-4ae2-aa1e-12921f5c2492','a7e6be3b-4f3b-482b-be75-f4b0cec9b46c','5778c91d-07ee-4fca-9b84-e234044b13aa','466d3922-5ba3-42de-9331-89115f5c64b3','305e6d2a-baa6-458d-8c8b-b4dbd3945ce2','a2bbbb82-d9ab-45a2-8144-4fd73349ea35','98b39fa6-d497-4aea-82d9-db021b3181ed','523b512b-c05c-4994-92b3-4510af1ec93f','c67aeab3-14f8-4e04-a79e-4b8d50d1b87e','cea9bfc9-70fd-43a5-878a-bebde032dd42','825e8151-5b91-4ded-aa04-2cd30e832b18','72982e46-981d-4a87-9f08-031759986716','87211867-53cb-4013-9072-686c6fc0e36c','0c1bcfb0-c93e-4fa5-9551-0bd6c04aec4c','75c35765-acde-479d-ba6d-04728eb2767d','5f4bba2b-73af-49b6-af67-5567ac9a53e0','d5678d45-88d0-4845-892b-bd7277c9d5b9','38919f69-a10b-4f8e-b7db-703b0c225848','86b71ea1-1548-4726-ac29-bb1fbd113ea7','2a9f657e-5f1a-45aa-89b4-81afe80efd2a','717c1198-fc17-4339-88fd-3f29d8648d1e','d4b6d31d-d4dd-46ad-8357-6c4dd59ac337','da64db8c-b7b9-4bcf-8a7e-91f4f6c7daae','08d34e3d-c9ed-4a9b-9cd2-08656d279f4d','e48f0da8-7c8e-4496-bc30-8179cba2163c','0ebfbbc8-e9e9-4839-9a40-be99d77d9723','8e3b769d-678a-4dfa-a98e-dd6c07431b94','9e97eaa4-d2c4-4616-a83d-00a7ff771e54','6617bda0-1ba7-49ac-a5fb-509117db368c','0cddde13-2e7d-46d6-9e70-4ed17a85184a','0ba40599-3ef7-47c9-bc1e-8b14b0411b03','ffd128bf-c365-4611-9913-c54f1181b2b7','83f7b302-8c3e-4d4f-97e8-ad9337929cc9','2d13de9e-5efc-4755-ac6d-6332c4672037','36aa6e70-b113-44e5-af60-08454813c161','cddb265a-75c0-465a-86c6-1d8c9f6b286c','0ed5e1b1-4688-4e2b-a4a6-7816871aabc8','c41fb431-a87e-4f3c-a1d7-21ececd8bd7e','2d3d0c09-df51-4b00-a31a-5d72cde74dc9','f2bf5658-dc66-432e-aea7-14bec1acd2bc','3787aea7-3fff-4771-ba77-6261b862946c','21d2ff10-2ec9-40f8-bbd2-c66b676be4c3','83002a15-255b-422f-8225-9ec05db7c56b','068f1506-a4a2-4813-bf41-65499fefdd6e','54faf053-8bd4-4827-b09b-0a4b35d3c6bc','8fe846ac-2e2d-42ed-9803-86cebc60a7aa','81eba0a2-813d-403f-bab8-faabec3aad7e','b3045ed5-4fd5-4453-b0ee-50579c4348ac','a8904125-9268-4d77-ae05-9b20bee8b473','2a9a6079-4d10-49b3-902d-6b6db7f2fc9b','f0e835b9-55ec-445b-9142-75a22a112170','b9bf869c-128e-48ac-9648-36734a4a7ad1','efab864a-e183-4665-82de-472dda57720d','d7f406a7-7208-4c7a-b4aa-eb7073b05da8','ef176a9b-1839-442a-ba3c-be6902f62b3a','e2f2639d-0f84-438e-9764-507aef6a2bbb','846e21fd-04b3-4e4d-985b-79b51c61bb8f','4b02c0ac-511a-4e86-869f-9fdc7495e5ae','a3627435-ff2c-4ab8-a05b-53e5362937e3','a321f4aa-9caf-4655-9f52-98a224521c3b','88bda0c9-aaa7-4b68-90f1-662eac5c5c2a','3ce919a2-4c1d-4cff-8faf-2554c68da365','e18549c4-8abe-4cd5-86a1-95f87ba41d22','43b5cb43-044a-420f-a41f-27813149e5fd','bb03a0c4-93f7-493d-a7b5-b152cdbecfef','917e7f23-f61d-48b4-bec7-9017f550e80c','c4dbf1c0-823a-491d-8228-44be6b7a068a','f6adc6c7-c4c5-49e2-889e-51e1482b71ca','838a12a5-a383-4e13-b9d3-182f30563f65','2e4686fc-ea6c-4163-a29a-3c094c3f8e63','0c82fdb9-bc9f-4b7f-853b-9700add8346c','d06e6edb-bafc-418b-a501-730f1a5fdc5c','0c1b4cec-1fd2-455b-8b9f-39b4af85c793','a2784759-e865-4073-be87-82d1ae204052','044c3513-e5fd-40f8-9c99-dfe19cbbe6aa','cd3d295f-37f4-4c46-9e12-778e095a165c','eb65706f-a718-4d51-ab8c-cc31f5ce0914','1729dac9-bbf4-415c-b21e-325ebf8119e7','f28281c0-9372-4586-8be1-88907b562899','a57bfaf0-7267-4ff4-96fd-4b616b210b48','63b0c85a-d1e8-41ab-a46d-0695390fe71e','358ad84b-1d5a-48fc-b7a4-81d23822d6c6','d6ad0ca2-801b-453b-a202-f476ccd03a92','fd2cb9a7-f6bc-458b-b757-a8254c22643b','ceea7b3c-fdce-43cb-b7a1-d7520534b8cb','458afd91-cb37-4acd-9163-9cb6588225ce','a907c695-8def-465f-b0f7-378af72b375a','40589b1d-842a-4fb0-b506-2199417f0d47','b7c28847-7cce-4310-b5ae-64f57ed82060','e702f5d4-f7d1-447e-8c30-0865306ed539','82204d78-0d9e-4d5b-be59-f48e1a5e5c25','e6d3479c-2246-4c53-95a5-ed8ecb74ffee','5405b114-9a24-4781-8d06-947d461bbf6b','7f06d9c2-ded3-43b4-8100-6512ace2b2f1','a75990df-1e16-4a5c-9861-9d32f0cff3eb','1daa19c5-c8db-4c3e-9612-21ff775906ff','ce6e966d-9ff7-406a-a564-7b27053461d5','8541ee53-5f10-4d62-96fa-3e13c98b074c','cedd1817-16e1-4384-9261-f76c43543044','57353cf6-3ea2-41c9-bac4-691e36b3d250','27d55848-41db-4d58-ab87-285c4e00cf26','2219544d-d0a8-40ba-a666-47a217637632','8e34ad63-bfa2-45e1-ac37-05bdb2969622','253c99cd-e83a-4e3f-aa82-29ac00aa0bc7','b617d43e-ef10-43a3-aea1-4c553c9f7fc2','ab372d4c-f259-4d29-8da7-6e9eab13de63','15eeb83a-4695-4b06-adbc-176f81a06093','681528c0-5766-4b67-a125-b6a14674ca06','90e5b4fb-d6c1-4b56-adf5-fbca09a3b7b2','94dcc18e-d9b3-41fb-9991-b30ae984df32','c7751581-1d68-470c-aaf3-8c05b4eac5eb','a68d8318-47b8-439b-b628-c81779b4f817','2e428f15-6e38-470c-9528-a83a81e1db35','6882d9e8-a759-4f72-970e-3536f2b5bc5a','641651ea-d203-486b-b668-777c001b114f','fafafe15-3802-4bbe-b9bd-31004fcde8d2','cf80aee6-d72e-4f39-9119-e5d5109cb0aa','2c2ab783-8a05-4aa5-b479-a02822dc2821','9039b08f-a758-44e5-8328-9bc61910f5a6','46f16144-785f-4c94-adc5-a7dad3687a30','96b6d73b-0122-470c-8179-a85cc7599439','9dd4195a-5de8-4c8c-bafd-66da2b9343ec','7189b9f8-43ef-47de-a736-61629dfd5bee','1f2cef71-ddc8-44e5-9904-8cadcdfaeca8','5ff5a4df-89cf-4c27-960c-fe80151aeec2','ea2012f7-3d98-4f62-8e06-7624bf30fcfe','c31b9213-4953-4c8e-8b3f-9fd3190b5ee8','9ef5243f-6d1e-4386-8975-683007c32e0a','ee8871d3-f262-406c-9e97-adde6abee366','3fbd3bdd-aaac-49c2-8193-872244f5d283','bbe13151-253f-4071-8d94-83e086385bb3','e3929293-7609-4ebd-8f2c-3577df3a27ad','f7ed5c65-dee1-4240-a0e7-c34486e4fc7e','15c7f956-1818-4703-98ef-b5fd8fedf89b','d1672987-5c7c-4931-b7c4-731035dfbe7b','a0fe84f2-2d83-4647-9d93-fcabd4e2859a','6c4b62fa-4a8e-4f04-844e-7142ad01c5c1','4f8b1fe0-7159-44ee-a84b-6d2cedda68b0','bf1e6899-e91d-4d63-b416-675a0ed2695e','c19afc13-88a8-4ed1-8f12-af045ffdf06c','906bf2d5-4f47-44b2-aa26-2d839f859986','2e57c1fc-9e84-4f18-85b7-6574697a2cb1','9e8abc11-9c74-4121-be40-fda642081de4','a6390108-616e-4eff-a9dd-52a25022bf87','65f2bfc5-e411-455c-be86-2b3f1ba631dc','d065b5b0-59c9-4226-9f68-663fe5356a52','90f4418f-1be8-4063-90b0-13ca265481c2','1c88b21e-2389-4175-9145-538c362227b8','f352646a-5b4a-4a2a-a8ef-718aa4b75f39','f9cd50ad-946c-471b-9f54-80d4da1fd70c','cf4391a7-33f6-498a-9975-de1140548499','0466153c-a72c-4a57-b170-bfaf87aa6542','87f6ca2a-f9a2-4d33-aa41-b48558db9dc5','5f3e4b07-1f6e-47fd-bb50-43647daba66d','896f951d-f42f-4f50-922d-3aa40451d975','00cae5f0-778d-4ec5-94a9-5f0e0407d826','d05328a8-8951-411a-98d1-9e4d76068916','96fa33d5-bfc8-4d7a-ba5b-a4c78253e721','9a675d69-aeb8-4343-afa3-c8caa8b7940e','7b841e53-2d38-4d21-b997-243079f3c0a2','e6b9692a-1a4c-420a-bd54-5906a53a0d2d','c142875e-b902-4cbd-9f11-f102bef692c3','e42c58c1-4d54-4760-9706-f3cdb7e702e4','516276ea-a1bd-4e1b-9fa9-ede05f8e210d','62ce231d-5d08-44da-bcec-7691dcdce123','10cb5e7d-ee2c-4a57-af16-aecbd54312ad','e2e04eed-7c05-4a2b-9940-9206ecfcc4df','1921f371-d997-4b84-8c4c-af85faf57924','354eb239-866f-43e2-8c7a-a872087438dc','c17a72ad-e914-4684-bacb-40a57be2244d','f04a1ab9-13bb-469c-9af7-2a1bd662c709','20d0b70d-fda8-4aa8-b3f3-2f9444799709','d563e71e-b58b-4e81-bcf7-73fc61dc635e','97ae5efe-94fe-4548-8294-6fba8d1cdff9','c0c826da-c5b1-49b0-aca0-1da06cec3c6c','80fad993-6c44-4aea-9f61-87100e460808','b0070298-9a28-4d54-8d97-b0f964514049','a08ec403-e2f5-4a9a-9ff9-8f19914e1c16','48067c45-4a3a-48e4-87e6-5f9e37cdd55e','b9cfbd2d-e8ea-4d03-939a-11c6ecbe2eae','cbef1bae-fe26-494d-a926-991071ad13e7','a31fbe4d-c6e6-4232-9105-40ddac6738cb','ddcf2b89-ed07-40fb-b104-de4cf31f4664','465af5e3-a412-40aa-aab1-72f68b0a5d5a','a8a80d11-4de7-4053-a973-a6b6e24ed2c0','7a2c4aae-6041-4220-95e8-bc6a2e29a832','4ab320ff-92fd-4802-a438-484013fec1b2'}}),'2601',struct('BlockId','00fe4c0e-9bdc-443d-929e-f5fbec842baa','SignalIds',{{'4af78577-99ab-44cf-affd-bb78ee1c9c96','b44702e8-82ea-473c-8cfc-c8e72c05b114','fc8a3bd0-b974-4866-b80e-c101785b72d0','fcd31d03-53f2-4b51-81bd-aecb4fbb7edf','6ce0dd2a-a282-4d08-b219-79ea85ab6b86','c44dd616-537d-4f98-b03f-5a2fd5211a89','817dc106-dbee-4548-8c78-f81a4dea449a','30459dea-8160-4fec-bbe6-67e9c6797f4e','919ebb6e-418d-4483-bfb9-07c33c74d968','50308916-c0e1-493a-8f7d-507dd1bb95dc','42b94309-31b2-4aec-96d4-4f1ae5167003','14c1c276-bac4-438c-a698-7210930d1482','fdcf97df-33ad-4075-8f22-79eda5c1558c','041af3d5-207a-4186-b748-ad47ba0904bf','498d264b-b3b7-4a13-a17c-1ef92b5c7e2e','5924fcbb-4470-47c6-998b-4f862a6362b7','e69d94ac-f895-4446-b3fe-fd7942b73c31','ef3c2faf-6516-4a4d-8282-569fefbe8eed','e2c7a58a-b721-4f79-96f3-5659395d58a3','5e5603a3-349b-4254-87cb-45eeafe99c22','af9ff53a-cea4-4e53-968d-c8c12ff4301c','b2f98a4e-e725-45e4-b1a4-8505ad0ed615','f72e1ea6-930c-4c65-be59-119738c7209e','c390c42e-f8b2-44c8-9ce9-d8128d358489','2d6738d5-5a1a-45f9-b88d-2ac018b43022','c752bdd2-1399-4a52-8ace-5ff5b5643139','b66ea436-4322-4664-826d-1bfe69742f16','74cca0dd-59b4-44b0-ad72-3ccf6fa07d5d','2ea5c387-248c-4920-9a4f-e1b75e58d31d','270cf674-efb0-4158-8677-ca88258ef130','ea915cc3-6e50-4b65-abf4-8a06f781a173','f552654c-3ebe-4773-aab5-ce1562bad898','55ecbc00-df81-4eb6-affa-2c48b81f9f26','0dbea84a-c734-4a46-a278-bc8ac1b77680','88b7dc81-3efa-4aa2-b057-330cbef75642','a7b8c5a4-2cd0-410e-8638-6d56ade3c7d6','bcbe8a24-0cb6-489d-b7f2-fa6ddb283d28','29d9f8c8-dd14-4165-be5d-7a5c18b283aa','7ea8c92a-ade4-4d0a-abae-fc1760fc8c03','3a0d261f-7132-40b8-8793-e2ee19673dcf','790a09f4-7e97-43fd-a99f-357211d43184','47f987b6-f7bb-4451-b504-891f9cb8e7c8','2534fbbb-60a0-4fc8-9d9a-3129ac08a748','9ea4ccf6-fc6b-43ea-b8ed-e63bcbd6717a','fefb8a3b-54e3-48d9-82ce-1cad449895ea','9aca53bc-f6f6-45a5-a961-f4848ff887ee','50cbfdca-bbc1-4630-9df7-5c90ae08e7d6','d4a53f86-4e30-48b3-a070-510a4282f02d','2fb41bc1-ec2c-4404-b771-763b1cbea142','e1064049-81bc-44b3-94c5-f90f66b7fc66','fd9c940d-e63a-4b9a-8a5a-b3956a132d39','80070ef9-784f-4e07-991a-3f029d24b3af','4fbc6b23-49cb-485f-911e-8a98909dd2c0','ba0c4eae-f311-48c8-a397-774c85045be2','5794d520-75b4-4db3-8ab0-a009d7a68d01','7569ac5c-728a-4fb7-9f7f-43b84be39f9e','a438f50a-de6a-4ed5-9793-e77e592ffbeb','6d16bb3f-6f1a-483f-a704-ff922481fc77','bb809cfe-fbca-4658-ba15-dbeada815d9a','8b69b6ea-74e4-4b1a-88a0-950c7e5f1641','76acc3d6-7fd4-4c8a-b6bd-010bd1a514b9','27a4b40c-f68b-4481-a13e-5208b7efd22a','2d7c263c-36f4-458c-92e5-0041443b4aea','ef055c16-61db-4f2a-8d24-6b21b4e681e8','60bff282-ef36-4b9b-8026-87eee72fe1ff','80f794dc-68eb-45a7-a414-f37c0d9427c6','d674e494-636b-4bb9-b433-3bd896838bc1','b39596d8-38cf-47e7-abd4-731bdedf3340','ad9049ab-838c-4549-a75d-e5adb6a034d5','eef73115-3b30-43bb-8240-f9d3677aecc4','8f5e49bb-70db-41d1-853e-1bb8018f4502','f4c58edd-d61b-42e9-9ea5-c1859f520176','5f7c8445-36d9-476f-9025-013bee28ed81','0604deec-9e83-4e8a-a16f-56e039387e6e','652ebabc-b629-45c9-b2f9-8508a05be1bc','d71d2d69-376e-461f-a701-2044a9e602f8','803ab941-4024-4b02-bc1f-0285179edfc2','459f777d-dca9-4acf-b83a-a85f23b24312','895d0f4f-7caf-4d32-87f9-5138a4c7c1d9','e5af17fd-e4e9-4307-9d2e-6b8b4a9c10f1','fffd4e90-e8a6-41cb-be67-5c89a09a3b91','415542d6-49db-49d7-bce4-cf60d5b30e96','2f8ef5ab-372f-4708-99d5-9976ec074cf7','4ddcc1b4-71e4-4505-b514-4b92684cb4cb','84082f89-ddb4-45df-8e30-bc20c66dd1a7','a74bb297-32ba-45bc-a82d-28853fe0c31c','ca4b24f8-3fb6-4a1f-b89e-623b37bcce21','643956b2-a34c-4295-b0b5-1a4032f85219','a37fceda-4784-48aa-9aac-43d585c2c6d5','b639258f-0841-481c-8708-9c2118ef4066','5a019a0a-5b18-4995-bb3d-cf3e5cc85a27','648edd8e-bfd0-41f1-8ea9-ac83183b5dd8','2b733cba-7da8-4a89-b0be-ca34b379a302','5b085248-b709-4287-b703-6bcdab504fe5','7dfdecd4-cbce-4bda-93ad-9929326bbd90','c80110a2-646d-45af-a6bd-e1872f0dad53','d4d1d458-caa2-4ba7-a9d0-2d22a4dcf1a1','91083598-856e-4a76-8661-30bef908a351','2933f278-9fab-49a6-90b0-a1f58e7629f3','8a93bc49-e52d-48fe-9a28-147227c07874','05c09b04-c2b1-4555-a53f-0b22f924ceee','79759d85-1b79-4489-ac04-78ac79aae6d1','7c35a72d-f96d-482b-bbd3-f254a1bf8aad','1cf99466-844e-4be8-84a4-140a693ebdb1','7b5fce70-5055-46ac-9687-97d0726a2a30','37d9a0eb-18ef-4b0f-b406-506c640dc87e','954d077a-4917-4d5c-86a3-a04eb7cb2754','fd6dd92b-dc3f-4068-9b35-0b25843e97d7','fb850260-ad7f-436e-abfa-8f6153d4e2fc','844e3dde-a860-4b18-9040-89d8c44e9819','e5b538fa-5281-4ae0-9a34-e6b385816887','4c9a7b9c-6f6f-424a-bd30-fc122292b51d','3ca4d12a-393d-498b-909e-17e509227d21','867e7474-e67d-4fa7-a93c-898614f7993b','f604089d-a727-4b65-a67f-21e497f2c342','881659ea-c95a-4cab-98a8-7e0d638332cc','a8acedd0-aeee-4dab-b2b0-58bb68e45c44','dd8837ab-84f1-4e44-bd29-1971f11ce39c','200b3787-db04-46e3-b891-c8b66f7b25ba','21234f58-203b-4723-a750-ff0e8f7cdbc2','abef4599-2771-4731-abb1-f75238f0f66d','4045bf5a-5679-4912-ac03-0a4b20efe406','7f7a545d-8abf-43a6-8808-71bed74cb28a','3a684168-6728-4e49-b14d-1a0601242532','bb912146-22cb-49b3-ba39-b3b15206dcf4','5535f324-92a6-4fcb-8f99-6315554d6ceb','293975ec-31ae-46d1-9ee0-ffa31d4ff7d4','b958f456-db7f-4914-a710-4eca84579d80','09c7e83e-808a-4f1d-b7cf-fe31af6e0e48','4ed05dd8-b442-4eac-b202-12a7e44598df','7edd9822-ed48-495e-9608-fc2837e08bc1','686c8df6-a928-42ea-8a97-8997b120ddcc','932d975f-529e-4ddc-89ff-7352124bcac1','427dc7c1-3052-4452-9ec8-36a073dc5288','e01789c9-a6c7-453f-ad98-bc09e310d2b1','d2b7a35d-ed46-4d40-9a6b-1c14864da093','df4e9963-1efc-443c-bfaa-20b40e41ca14','d752e6f2-60c6-44c3-b665-6c44c4a1722c','63378fd6-6d3b-4060-b102-4e211909f8cd','d3a6ee8d-7468-42ad-bf6b-546885e4b907','7266430e-23d2-43ac-87cd-8409e5fe11e5','5e717a87-c254-4fa0-acb0-4d68803ad9d3','ebbd9276-cfb0-4e62-9a7b-e133dfa14f43','0cfb5f06-0d6e-4b9e-9633-e2921615c338','a3b9e667-5ef1-4318-b7f1-cb9856f6cb00','cb269ead-bb02-4906-84c9-f41c0fa898c7','363a4e93-ba35-49d9-b98b-ab1e326b3444','887c111c-7811-4a64-a9f2-4dd60575bfc4','c3d3100b-d78d-4211-bb03-83a5ef665171','6498927b-1bf1-4a7c-bc6b-42fbbbc26167','e12882bc-f788-4cd0-9dd1-1aea57a046ce','00ee0042-d2e0-4e3d-8646-45a41434d703','2d06a604-6928-4e70-810e-49c13ac57c9e','ed74922f-157c-454c-bc4e-572a375b0e75','221ad922-8bae-4dbb-a9fd-a5ef9af2ac3b','895d38c1-fe33-43f2-8151-5082982269e3','e59a09fe-62c2-412f-b5ca-7c62c10f8c6f','71ed8775-5fef-4de1-92a8-8d2008b78a28','c3003d31-b49e-4e0b-9e69-62e67a0d88cb','3936a8ef-7c11-45a7-b425-a2dc995f9bb0','a587d09d-940c-4c8d-acc5-7105be9e4718','3da73a1c-976b-4465-a6ac-327a66ba0c0e','b533f75a-b9cf-41fd-b7a1-1aebae03e2df','c5b61f16-3e3d-4d4f-b2c6-0721c7f16a99','7dc2a3d0-f0ad-4426-897d-2e911e16c45f','3a0981e3-f3de-4045-ab22-fb104c94b41d','b6734df9-7844-4325-b386-bd1383e1f837','f8a5cb1a-4294-4cca-ac06-229409bac371','b02beb2d-4173-4111-9820-5c9b63c1c67b','1ecdfce9-c797-4f91-ae09-e6209bc1bbd6','babf5397-b992-4770-8a60-7ed7e6be5bad','4baa7488-a395-4e69-8e5f-b810dedb47ef','ea5033b8-5b51-41f7-977c-b24f1415e621','bbda337c-9d34-4955-b5ab-715b1f240fa3','1a66ed8c-d4ab-4553-b2eb-650e95a8d2cb','dab9d818-ab45-4f68-9e5c-53463db71dbe','fbdcd41f-7a7c-4b43-9805-01b34e2c25de','3e034651-1ca8-434b-8973-ad10aa2b206c','7bc372c8-ab10-4b62-86dd-68dbe7de8f69','54cee070-c5f3-4c95-b568-8b3ec629b34e','e1b1a998-fc3b-4977-bcdd-aa6f6421fb70','30bc3ae5-bf77-4699-8980-e68be5422b0e'}}),'3',struct('BlockId','189d5407-1534-4d3f-8c8f-29d0d30c5488','SignalIds',{{'7603f1d3-8e36-47bc-b737-c3a14e4f2bdb','13caad75-2fa7-44e1-83d0-c93884482ff7','ba8ff35a-2dd0-463c-a93c-aed2e8b16826','4f4274a2-cac1-4807-b06c-23c385bc3c01','cf9b38d8-e7cd-4582-b04c-3b740ad36a67','53a510ec-fea6-4c36-a3db-15d40d5465d6','52ad531f-b356-4b98-9b15-ac6512a72b44','ebd11de4-ada3-41b7-8951-a6a583ba8332','21108067-8ecd-4034-af77-f2be947a5bf9','728a86ad-ee7e-4470-8043-853d06e5762a','89d67a9f-f5c1-4d06-a67e-ebb046c8e34d','ae8d6440-7946-4b36-a246-dc03fdb497e2','6ccf919f-c114-484e-aa8d-a623741d9e13','5119f3cb-f3cc-4ef5-9b6f-b3e4fc81e6fa','59e7fe00-b3c5-4de2-b80b-9c014d037412','513d3c4e-1235-4d36-8667-54e3e83ab4e9','a6177a7b-608f-4a36-8292-578a69123e09','868c1203-027b-45c7-9e9c-6657934e48a2','9237f211-749f-4b6e-849a-76e478c8e66b','71dd4c62-d529-4fff-ac41-0822420c8640','351e6ab5-4e10-4180-9d37-478f302f9f27','d0c141f7-7f19-4837-ab02-9514cc6e0859','7613534e-2be1-4a72-8590-bdfccecd2dc2','e684d649-0c66-47e4-bfec-1071a99f2f2b','ba7ff62a-fa96-45ca-b8c1-3cdcdaa1311c','ae99f73d-43b4-4531-b5a1-6fe353d0f72b','94a7d6d6-70d1-422d-b3eb-015ea980a1d2','d7b9b511-0b58-494e-a815-b721173414cb','62994ed8-3964-4221-9126-e04dcd67c089','37398f04-44a5-40db-ac18-95b02175a359','daf273b5-b7e2-4036-85fc-c7c42fd2f9ec','02e5f87d-cb11-4f49-8956-a4e1e461ff42','62524d82-3a78-4b29-b299-3bf46e4e33fc','9bbeeaa4-0880-48c6-bc69-67c48bd46129','4d3e1888-af20-4028-a496-4e02c52a6db6','d1e78034-2554-4478-93f6-dce3f86d999d','29a82bd9-2798-4bc1-aa4b-dd956a6dbcea','5fc76547-a1ea-4544-b847-0e68dc895db2','f712e83d-bbb4-46e1-bb2e-7a0033af1f93','6279295b-555a-41a2-b7e1-f46ee5a1d15a','c6e4781d-5c11-4f50-a433-439bc086c719','1ede554a-8eb3-4df2-b0db-eecf87d9cb7f','7a88793d-25e4-460f-9ddf-4ea44a20b127','be9871c5-43c7-4c12-a848-d6b03441cd6a','719b97cf-0037-4c34-9ebb-77df580626c9','dbba3b5d-c9b9-48ab-9503-781155fecf10','4b941849-304d-4a0e-bfff-6051fb1ae26f','07a314fe-455d-43e3-a415-d8670d7529ec','d325ab1b-91e9-4b14-8e2c-0399a190b825','ca8c4151-cc10-4538-ac46-8fda666d68e3','1beed3db-da84-48da-a2fe-f919e94474e8','a53ead39-59c2-4306-a50d-74f10ed1be0a','7aa41fd4-2816-486c-aede-b1166d979b67','b472dd1b-d931-4843-8175-0a4c4707077a','de3ed365-e66e-4d52-a120-5fc71736b6a0','9862361a-eea0-4201-8e96-9a203e3bf6ae','643e850c-61a1-47f8-9dfc-ddabfe1a7fd5','802d4a86-1087-46f4-bc32-28cb9f7994bf','9aba9ae9-e4f3-440b-9622-bbdc3bba320d','0c9d98dc-281d-4762-bbf7-e0b4354884ac','068d42a9-c246-40a8-b3b0-eb4433a3a1b8','557d34dd-61bb-423b-b419-94cd59bc665c','c1c73360-8ed1-4741-9da6-fce539b91436','62ff4983-eb0c-43a6-abdb-653402d8c632','f6fc47e0-43a8-4ccc-a682-6b89672a20c7','894c759b-3024-4d4b-b146-acbb93e3da3e','56e406bf-8dca-48fb-8e0a-473bc6d76c6f','b26bddd7-e93f-42e5-87d4-421e6294edc5','eed44345-f0ef-4d4a-b857-11fb06335e45','eebdda50-1124-47c8-a980-6d6d6b227896','1b6863a7-b6d7-4d63-8e40-cc713568225c','31c57672-025a-4bd0-8c5c-4ae3735bf1b5','26d725e0-9853-4a7f-b866-0125700fbd7e','44b28be2-eb80-4392-9d8d-737cfaeddc66','6c8f56b6-76d0-4d94-af1c-1236b515ad0e','7641116a-163f-4b57-a6c6-a13d0805a7fa','95027ae7-4513-495a-9905-280f40b7b7f5','bf26071c-2690-4f70-a482-9e11776247c2','fd552f46-60e5-42f9-a325-2916bb239a08','f87a255a-4e6b-48a8-a332-0ee0d15f8d75','c43dfac2-e751-4036-b977-3f107db1a5bc','169def89-1d1c-41b5-8d99-57b7945577f1','c00b02ed-ce47-41ea-b0b6-f42d8c96750d','f7f00dbe-44b1-4566-bf99-b63c94010ce1','27e1dc93-df06-4724-b3f8-964a45e29ff1','3af8eef2-b308-4273-bb98-2d2687c66da0','57074f8e-d8c1-44a5-983a-3bd9a0f7d73d','523b6219-3480-4819-bb81-8abdf8e7a407'}}),'3609',struct('BlockId','cac39ff8-1014-4c6f-8efb-e0af7d908f52','SignalIds',{{'2063a541-1168-4f3c-8434-b1ae1b5e565a','6d956c46-21dd-4d6f-bee8-9a531be294e9','9c8562e4-defc-48b0-b894-de1a8b48766d','87df9953-01ad-442d-94d2-a90adb926c69','4b3aa4c1-ca74-40f8-b5cb-a5821be7594b','26577ee9-e37f-4a07-b3a5-f0b2555bdd20','0e6b0ed3-b9ee-4dc6-8f76-11ea9a9426eb','086f9bfa-3db3-4bc4-b47c-e8df885bcb0c','970d622e-a606-4fc1-8e9b-6e7abe5290ae','4e4d40cc-712a-4361-b89e-c9dd8494365a','5f991e17-9fce-4af8-b0c4-e8bb9a0fcbb6'}}),'3610',struct('BlockId','bd3df64f-c853-4bae-8dde-c64854b03ebe','SignalIds',{{'61184362-b6a2-497e-aeec-1c9fad7d916f','5fa47b1e-1ac1-4cca-a486-149598553fdf','6e9267cb-67d5-4b8f-846b-fce9f1b4dc47'}}),'4',struct('BlockId','0b82c8fd-cae0-4d17-8c76-acb7538206d6','SignalIds',{{'550b4886-f5f7-4659-957e-226cb2ba261a','90dffed1-b471-4292-8163-9fbec1af987e','93e9b1c0-9513-4f91-a825-6c5cef114d17','a0412f46-2ac1-497d-9eba-e66b834dc2e1','a2839e15-18f0-41db-b553-fa8390e94806','7384be57-f228-4a40-9af4-d1295a408e59','eecd652a-5e99-4532-b325-dcaa5ce88090','a3e5eb93-c4f0-4e2f-866d-d6cbe020caad','898fc471-510f-41b6-9dee-f9b4e267e9fc','4a334083-f584-42da-be08-927abf88865a','7624e54b-1811-40b4-a3fb-7b38b392c5b4','06ac65da-cc93-4134-a97a-06ce0a826e43','12842ae6-db5d-43ef-a229-a43c2a01c23b','967c5edb-e39a-4141-803a-8e55f2d89302','890fb909-d74c-436b-ac1f-9d6882f5a51f','950c4c37-edf4-40e7-9d7a-207a177edc94','e86bc5b6-8898-4f57-9afa-5df2d80db851','5026454f-354f-45c2-b30a-f9a8152108e7','ddb8b6d1-2e09-4482-94b4-cb276b810436','96354517-d05d-4566-b95a-9f3e43afe59a','725527fc-6d3c-484f-bada-4e90813c00ce','55e85afe-68c1-49f2-a2e7-5920cbb7b7cf','89fae035-1463-4c16-b6f1-ad9c92e9c606','698bc418-2281-4eb0-bb6f-e9fdef440322','d35b541a-cad5-4c0a-972b-51da497ed932','2a736442-fabe-4e5b-ac3b-e88f4c8a1ca6','e06c06ac-099a-4f97-90a1-d116cf2ceee3','68ced3a2-bafe-4774-ab6f-37c4655289da','9be36a2a-167b-4795-a4d1-210e60ea3bf7','886f179c-fc9d-47ff-9897-fd40782d0779','4b2b1be4-5333-43a9-8d37-a2d018a33c2c','de33c6da-a000-4773-a57b-982968d461a3','51a11165-48df-4960-a180-abb7852adbdf','59507665-680e-4995-8f65-3875c03db80f','197f9fcf-9477-4d79-9fde-fcd763026307','71736d90-dffe-483d-aeff-6802131d625e','97265b4f-4cee-43b2-a7cb-6ecc2fee221d','340fc7ec-bdca-45eb-b97d-df996c0d1143','4bbc8bdf-7817-40be-8ff8-49ba7f7e36cf','53cf5376-ea06-4124-9c07-e1f4b09d37d1','3d8232b2-be22-48c0-b6f9-3b76797be9c4','6b917c9b-4c0e-42be-9e5e-5e85d93ce71d','142f14e1-e4f4-47de-bf1e-083b4feab2d4','68641e10-c86e-4ecb-9331-49c75437886d','542e0c1b-6563-4b36-84f9-4040c1bf2737','84633952-c8f7-40d8-a215-29b1e5e91f6a','2af09684-7708-48e1-af8d-702634dca86d','f38f7f76-cd35-4f8e-8def-62401723f8ec','2eb50915-2b14-4009-b80d-0fab6cd103ee','7f1cb3cc-4afc-466b-b9b9-5ef57b310f7f','9642c5c9-9730-460b-baf2-c22a41b55936','e0752c2d-e59f-436c-a0f1-95c1f01b2344','25bf23b0-dd59-4d41-95a8-1d2572f78bee','5f6e29f1-cd17-4401-8873-854b5f27ef8b','e9d8e0b7-eb51-4850-9b17-0e0dd43ad398','585dca6c-cbf6-431e-b75d-1b5f565b0d0e','295c69bb-d8e2-44d2-88cc-68a4b5aaa38a','6be83899-6225-4e7c-bebb-6847e381f0e1','4278a4e8-d80b-475b-bf3d-0a1e9dd2ce63','63693b94-b736-4b8f-a174-0e3efb4fa238','ff13d461-d520-4884-a487-6e65efc91504','8050b67a-ca59-4ed7-8177-ae044ea6b6b0','e2fa4d7f-1956-410f-944c-3a42689a3c38','37ffde88-2842-4577-9231-96ae98e39950','4dedf8b4-a511-48df-af46-4cf623f22dd9','2055155c-0f86-4135-b5d6-3f6fc33d2ab4','96b8e5fb-36f9-4f17-8c91-507e3386b39a','9f1afc40-fa76-44ab-b0aa-fc5a601dd690'}}),'43',struct('BlockId','6fcfaa63-0a10-4e36-88cf-f3d5dd8caa07','SignalIds',{{'47698925-1808-425c-bca4-a35bb8269ab9','7ff98473-86c8-4288-ab46-02fb0c48f1f7','4880dd35-44f9-4e9a-95bf-7c939102cfa2','0bc47c38-e38b-4105-8b1d-7f2f571ca367','b2f248b5-ae2d-4368-9eab-a86eafdb77e4','248ed30e-9a54-4e25-81d4-e6dd36a10fc3','7d7adcbb-f450-4164-9bf1-7aed10cad8ed','b00a4ce3-bc87-468d-8c50-911830a4bf3e','ae0a3348-5dec-4ead-a7a0-674eebbdfe06','5bfc7741-8ac1-4f42-b1c8-3fb39f4f7491','064ed7a7-f530-4e0c-ac06-8f18f3f6f1aa','43792134-813c-4750-8ed7-61f3d02dd889','03f75be6-c142-4d5c-a129-4cec7128a883','7a145475-8e83-4962-888d-fc044daa9919','f3bb0f6c-2895-466b-a26f-9c9e15abac05','a2823f13-c40f-402f-93e1-c15c94da900f','c3d5be94-857f-4431-b9b5-e2a91bb2242a','f7127502-e47d-4821-add8-65f25f15de37','a8510e41-840c-4a37-8f77-f55e798da1cf','91d3dbd3-feaa-4207-a97e-4179e64c93e9','170a8667-0ace-47c9-bf14-936ed702c245','96842592-a82b-4788-baa8-9e0122858aa3','8dd04f80-12b6-4414-9b4e-a9da58e91bd3','3fd598b6-4491-483d-a8db-df687b135489','5086743e-bee2-494f-850f-adb23a7ed123','ca72b7a4-7d93-40ef-8752-e3eb000cf00a','618cc274-12a2-48db-8a57-92caec39b96b','1e55cca7-751d-4b14-b978-77e86d3c02ad','67790ec6-2fde-48b5-91e3-5fc74b89b244','69c441c0-6714-4c32-b5f1-195df51f9db9','d205bc56-6501-4210-97ba-c1fef095d383','65c112ac-cabd-466b-b1f7-944282929d83','10024e4b-5bb0-49b3-b89d-aa0ed781ace1','59d50ff5-2489-4e3e-9c33-b1ee99bb2b29','4c238628-2474-49d4-ba2d-42311c6d3209','629cfaf8-c0c8-4a93-8468-ee4452b1c14a','500be14a-5c9f-468f-9f1c-9bf7deac4ef0','d6689070-81a0-4603-b5f6-dc718defb70c','3d3d350d-4cb2-4c8e-a633-5560ad008155','bcd7e5a6-39a4-44d7-8409-910bd377376e','582700a4-2391-422e-85b5-614e98aa502c','508a0e3f-45b5-4c40-9c2d-c172f4480bb9','5ab6e6ac-b42e-45f3-8e41-0e32db950700','275e2748-3267-40d5-a4d5-3e7144e0a4a1','9944c3b0-f294-4fd9-b378-caeeb6ecc26d','ef6d0378-7977-46b6-85e9-bc423b8fcc40','dea42070-0f76-4435-88b3-fb58de0f5fae','7f4af973-30f9-4926-9540-fe88a7d88346','2d9dcccc-e297-4658-8170-a65cab3dc204','c4a3baae-32a7-4724-afe9-20b8df65f73d','a81d75ed-7134-4c49-aa16-d56b6f5d2c73','88339940-07c9-48fa-8da6-fad0c4dc2877','3d07abb5-23cf-467f-9ef2-768505b6225a','27b9d9e0-7a9e-499f-a1d1-1efca6f127ea','05388ed2-d623-4a5c-81c4-ad211d0fe2a6','19969f95-5beb-49c3-88cd-acb97c30b62d','de5b8424-280e-4427-8901-e94b286f9305','3446e292-c53e-4b0b-901d-dcd43449e39f','0ae4c8b3-bc66-45a6-8b8d-3f2446b4c9a2','8a54859e-a482-4bf9-a3f7-5a1284ebe25b','58c1f556-959b-4db6-9579-10a5d2c6b9ad','8d601e86-121c-418f-a6b1-7cc79cb062ad','21afb3b5-810c-4fc7-b2d1-6c7c61aba301','1914e5ec-5ab6-4324-a4c6-36f7d01c43e1','8bcf4b06-7924-484a-b3a0-9bafffb8951c','f0eba240-80fc-4db8-828e-fbef68fbeb63','813c678a-8518-4b1a-8c03-b370956bd652','2e11b84b-ae72-4b35-b706-4c906df3877a','99e4a026-2a90-4b64-a745-9b1f5566c2bf','106b8599-4f8d-401d-b4af-f20f07c25b5b','21a2ef4c-d996-49e7-8b58-e7c68c3903d8','7c844853-0d92-4d24-9987-5c1070702fb8','25025917-368e-41de-aaa7-d7bce2cb90c1','14365f7e-0148-4cef-ac3d-2167d7d5ae70','ca7854e9-f039-4995-8bdf-b1e6d7195e50','c29878bf-3865-44f6-ae35-b0e7ac16e72a','8bf7dcfa-3253-47bb-9e7c-d17874150b55','81fff3c6-e0ef-4f2c-9f7b-2cfbc448a696','5ed8e2e9-7dd4-4144-8613-885c8e4c229a','7e68e1ae-22fd-4c7b-9762-b8deb17f806d','a9f70856-74bc-449c-984f-d13aeabdb517','770d9d62-6142-4a5c-90b0-b402c982b469','e1f5391b-eb4c-4fe9-9499-73dbdf4189f0','78fba2a3-dacd-427c-9ec4-2192a957f5cf','4022f901-343d-49e0-a5fe-b1a7e7375df5','35069299-473e-4c4e-9842-9fc814e185d7','fe2a2268-d1b9-447e-bc79-338d3321da6b','1797019a-4a94-4ad0-a5a3-9e2916b04b32','10180bf7-b92b-4a7a-a3a6-98a8b4b533cd','e35d08a6-c7ba-424e-bca7-f6617e439790','710ba258-f230-4a61-9055-40e6b5e53dd8','ca7254a7-7ebd-4ee0-8fb5-4870dd8d29e2','7d57a9cb-5096-43e6-b4f3-a3babe300e6e','90fa89c4-1ef4-49c5-a7f9-21f708fcf060','0a34feb4-4383-4e6d-804f-038523980cb2','54a4d812-13e4-4612-8b5f-9d80cd9fe275','b3152e83-3c7a-4b74-a369-c1a2197c0cee','b22e4b11-91c0-4376-9100-89e09c59c537','5dce59ac-7574-4a75-bcd9-58a499a886f4','de7d62ba-694f-43bc-8a1f-648ac5d80053','1b886dc6-2f20-42e4-a549-27391adb76d4','6839710c-16dc-4b65-9074-ca83c1c7200b'}}),'68',struct('BlockId','1824beb4-a74b-4478-8efc-bc612d452223','SignalIds',{{'1b02cb7a-4e31-45b7-8660-e7e1968f9ecb'}}),'79',struct('BlockId','b0ad6007-c3db-4cf9-ac26-f3769d8a7728','SignalIds',{{'c44a09df-9172-4b5c-93f2-f91166640fe8','52ec159e-0aea-42b7-ac31-5cb593721378','701309c0-0104-45a5-963d-d014242b0661','506706fd-99ef-4ef2-8f48-9d0ffb70fd65','58f2a182-bfa0-4507-b418-9dcd6116945b','0de90622-3b27-41d7-810b-de35b04d0cb2','3e03cf24-9c23-403f-8c87-ecca832daf2f','dcad9876-06f0-468c-b559-5938289337cf','493c96ce-1b5a-442a-b097-368af4297e62','37f87e88-f3ca-4147-92cd-0bd69b773c34','97bff1af-4a42-48b1-9235-b2739e07f883','d4f0b5b4-d530-45fa-a4da-2358a247e7c3','e8eaba52-6f67-440f-8f87-c13294795dc8','3115dbd2-af4e-4ea1-9a7c-0ebf302bf60c','1bcd1a12-3c70-4ec2-a719-cce9c94af964','fbdb2c46-2614-4ea8-bd21-177c56b32d62','21a27ab6-3082-4a63-93bb-628a88ab1934','2b74a90f-6563-4723-8839-58ab5d02bbc7','8c1b4999-60ec-4c90-91a6-6251d4d91b08','4849a16e-d356-4bcf-8658-7a79a6e4cab9','e4046c70-78c2-4ee9-81ca-22f2bb54db37','94a30874-40f7-4ba5-b1aa-38ab19340ee5','585aa150-8658-44d6-8e85-9271bad74393','e6f3aa67-1dd6-45d2-a89f-346e46b55aec','a3b20955-7d85-4c5c-9881-f0ddc0b100b2','a937ff4d-b250-4a3a-8fb3-203a051be92f','18c86531-b92f-45e8-94d6-cbe1e3c50354','8f5f72d5-317b-4fce-a7f9-693241b74b99','7c0919dd-10a9-4cca-8e5d-6826c6d54bcf','043a742d-7438-4722-a9c1-ac15e551f5ba','1dfb8ca9-d9e0-42ae-b69e-5a7fc65b4e30','cd39be96-9fd4-4852-ba60-93b08ae54958','e0cabcf9-a2e3-45af-82fd-ac094d5e8647','0690c6af-dd13-4e92-9dc1-c1fe0f3f0f57','57b9bc19-a8f4-45d1-9411-322a4025a2b8','a04fc7ba-f6f8-4e86-9b9d-7089eef7cda1','6c37faf3-0554-4b57-9311-e231c2076c60','e84c965d-093a-4cda-a5be-f08ecb452a7b','b86478f2-0f06-4fe4-a60f-c3a2e463468a','f4055928-3103-4e03-bda6-81f342abd8a2','db8398ca-01df-4850-961f-8e44db4aa5f6','5e9ed76f-3bf0-41b8-aa78-076ed642f031','713ad1cb-04d2-4b01-86a6-88e051473e03','9c38ed7c-51d3-4fda-a065-52703fda8fa4','7abcde11-ab31-4d1b-9807-1846fabaae48','09a51767-c02f-4ead-9156-f44a635a2c6c','21f92d23-5522-44cd-9290-d3cbee37c628','ee95f5f4-7152-4d9f-8c42-0e4deee35d78','02587bd6-14e4-4aab-adf4-69ff8b7e7b74','8f257aa1-f142-4e73-9705-a40d74509c40','19a73470-6a7f-46d3-b784-8419320a75da','2a6c056e-c082-41d8-8cfb-f733d4579b67','9fc74eda-0f12-4aec-abc0-fe2286dc12a8','e0bd967a-f0cf-4a20-bbaa-8b56cbba2f6d','f94e5e1e-3b68-4960-a3fc-412c0a089475','9b5b5d1b-50ca-4529-9604-f814d4e41fd2','a8e8e774-f044-407f-a3b0-cd9fcca1f62d','ba1f95e9-2bf8-48fb-9168-f9075c186853','7ea323ad-bb73-4204-8680-cdab683de12b','8e08edb2-9c6b-433b-860d-93fa851d2395','bb575d71-faf7-445e-a0aa-2a43c8c64241','88bf46db-601c-408d-baf2-2061561a48a2','e85c8a8a-ebf2-4066-a513-f16157a4ca83','80077b27-87f6-46ad-a3d9-1f22e200d331','02aa6618-7aa4-40d9-8dfd-5bfe9a379617','652e7169-f6cc-4d27-9aea-3a3756b03eac','09188da7-36d6-474f-b574-221c3ebc41ca','1c4a4e1b-c430-40e8-8846-2f51a9de5389','be7106ca-d2ec-4876-b717-1d5c2512aa2f','3cd6d13a-73b6-4a2b-9ee4-1af317c72d3e','c1d8a3b6-0640-41b5-9c15-5f99560c887f','ff777991-f8cf-4f95-aff1-7f4a48498818','f23d68bf-5542-4474-9b82-007ffe6b0db1','f04b9c32-1527-4c63-a63b-4c10e8865782','3296807c-5a51-4c4b-9c2a-8f8a3846d9b2','8f05ea6d-5bd3-4bf7-b03b-498ad251f5fc','54fedde9-80b2-48fe-855b-3faa4497015f','8e25dfa0-16f7-48a7-8f11-13c93a30eefa','20ba1748-f28c-4178-8b33-361db220f29e','0d49a5dd-a527-45e5-b6de-b4f007ff21e3','87522574-6efe-4289-b67a-1f19dc87fdb2','98eee306-e7e4-4be1-934d-34ba67e02e47','ebcb05d6-8dc1-4663-b8a8-b08a1c74d7be','4e155d15-741b-4d45-b93e-f41d2518a721','b34650b6-eb18-4e41-859e-05798ce04805','bee2ca44-881a-4ce8-84ab-75c8cacbf7d1','5bab04a3-1a72-4bd4-b1d8-3b0b58e8f161','ff83e4fd-b607-4606-ac4c-ed68099b700a','19c30927-2916-4720-812d-7db07dd7e35c','b6dcb784-dfa1-4dd7-b59a-19db8f5aac7b','fe5c8d87-b6b0-478a-83f7-4801a744cf74','4e4f62c1-a9b2-4057-9e65-49084bca5042','227c1dc8-b281-4b30-a8f8-92bbae076463','fc4acdfe-29c1-491d-b141-f9d2ff0ad663','960c01b7-e657-4dde-ab60-7d42a0e331fb','65ddf4ec-5a23-418a-bea4-c9904fbab09d','d6bcae28-0856-4d35-990e-e1f3002508e3','7c15173c-bee4-4580-a315-923a17a746d8','6a2891eb-8381-4e04-a5b8-da1d7314fe73','21e39f08-5232-4cbc-8eaa-e2a42b8ad4e1','25f0c8e3-2006-4a87-aa30-056ced5568f3','254d7d24-4ead-4036-8824-5a010c6ae68b'}})}  Creator=Cheng  LastModifiedBy=Cheng
settings OptimizationCC: BlockReduction=off  ConditionallyExecuteInputs=off  OptimizeBlockIOStorage=off  BufferReuse=off
settings DebuggingCC: TasksWithSamePriorityMsg=none
settings HardwareCC: ProdBitPerPointer=32  ProdBitPerSizeT=32  ProdBitPerPtrDiffT=32  ProdLargestAtomicInteger=Integer  ProdWordSize=32  ProdLongLongMode=on  ProdHWDeviceType=Custom Processor->Custom
settings ModelReferenceCC: EnableParallelModelReferenceBuilds=on
settings SFSimCC: MATLABDynamicMemAlloc=off
settings RTWCC: Description=dSPACE Run-Time Target (for VEOS on Windows and ConfigurationDesk)  SystemTargetFile=dsrt.tlc  GenCodeOnly=on  MakeCommand=make_dsrt  TemplateMakefile=dsrt_default_tmf  RTWVerbose=off
settings STFCustomTargetCC: TargetLangStandard=C99 (ISO)  ParMdlRefBuildCompliant=on  ConcurrentExecutionCompliant=off  CPPClassGenCompliant=off  GRTInterface=off  SystemTargetFile=dsrt.tlc
settings GRTTargetCC: CompOptLevelCompliant=off  ConcurrentExecutionCompliant=off  CombineOutputUpdateFcns=off  MatFileLogging=off  CPPClassGenCompliant=off  UseToolchainInfoCompliant=off

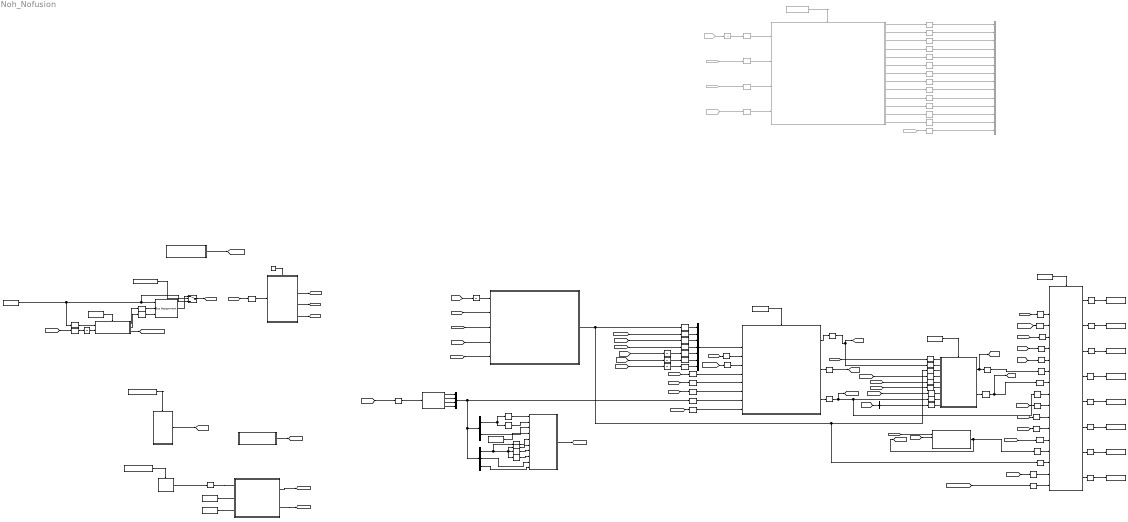
== system Noh_Nofusion ==
  note: UDPReceive
  ACC_FD1 : dsmpblib/Data Outport  Priority=-10000
      settings: SourceProductName=dSPACE Model Interface Blockset
  ACC_FD2 : dsmpblib/Data Outport  Priority=-10000
      settings: SourceProductName=dSPACE Model Interface Blockset
  ACC_FD4 : dsmpblib/Data Outport  Priority=-10000
      settings: SourceProductName=dSPACE Model Interface Blockset
  Bus Assignment1 : BusAssignment  AssignedSignals=CSA_NODE.CSA1_MSG.LTurnLmpSwtSts,CSA_NODE.CSA1_MSG.RTurnLmpSwtSts
  Bus Creator : BusCreator  Inputs=7
  Bus Creator1 : BusCreator  Inputs=4
  Bus Creator3 : BusCreator  Commented=on  Inputs=14
  Bus Selector : BusSelector  OutputSignals=EQ4_LH.EQ4_LH_ELEM,EQ4_LH.EQ4_LH_HDR
  Bus Selector1 : BusSelector  OutputSignals=LSM_HWA.RoadWidth
  Bus Selector2 : BusSelector  OutputSignals=EQ4_LA.EQ4_LA_ELEM,EQ4_LA.EQ4_LA_HDR,EQ4_LRE.EQ4_LRE_ELEM
  CAL : Subsystem
  CR_RSDS_Input : Subsystem
  Chassis1 : Subsystem
  Common1 : Subsystem  Tag=<DSModel=3_'Fusion'>
      settings: AttributesFormatString=<DSModel='Fusion'>
  Constant13 : Constant  Value=P_BCM_TurnLmpType
  Control1 : Subsystem
  EQ4_Lane_Pack1 : Subsystem
  From14 : From  Commented=on  GotoTag=IfVIEBus
  From15 : From  Commented=on  GotoTag=ifVSMBus
  From20 : From  Commented=on  GotoTag=LC_Obj
  From21 : From  Commented=on  GotoTag=visMsg
  From27 : From  Commented=on  GotoTag=IfCANBus
  Function-Call Generator{1,3..5} (4 alike) : simulink/Ports & Subsystems/Function-Call Generator  sample_time=0.02  numberOfIterations=1  DisallowWideOutput=off
  Function-Call Generator2 : simulink/Ports & Subsystems/Function-Call Generator  sample_time=0.1  numberOfIterations=1  DisallowWideOutput=off
  IFC_FD{1..3,5..6} (5 alike) : dsmpblib/Data Outport  Priority=-10000
      settings: SourceProductName=dSPACE Model Interface Blockset
  IfRFM_LANES_In : dsmpblib/Data Inport  Priority=10000
      settings: SourceProductName=dSPACE Model Interface Blockset
  LPV : Subsystem
  RFM_Road : dsmpblib/Data Inport  Priority=10000
      settings: SourceProductName=dSPACE Model Interface Blockset
  Rate Transition{1,3..46,79..92} (59 alike) : RateTransition  Integrity=off  Deterministic=off
  Rate Transition{61..78} (18 alike) : RateTransition  Commented=on  Integrity=off  Deterministic=off
  Selector1 : Selector  InputPortWidth=4  IndexOptions=Index vector (dialog)  Indices=1  OutputSizes=1
  Selector2 : Selector  InputPortWidth=4  IndexOptions=Index vector (dialog)  Indices=2  OutputSizes=1
  Selector3 : Selector  InputPortWidth=4  IndexOptions=Index vector (dialog)  Indices=3  OutputSizes=1
  Selector4 : Selector  InputPortWidth=2  IndexOptions=Index vector (dialog)  Indices=1  OutputSizes=1
  Selector5 : Selector  InputPortWidth=2  IndexOptions=Index vector (dialog)  Indices=2  OutputSizes=1
  Selector6 : Selector  InputPortWidth=4  IndexOptions=Index vector (dialog)  Indices=4  OutputSizes=1
  SimBCM : Subsystem
  Software-Triggered Runnable Function : dsmpblib/Software-Triggered Runnable Function  Commented=on
      settings: SourceProductName=dSPACE Model Interface Blockset
  Subsystem1 : Subsystem
  Subsystem2 : Subsystem  Commented=on
  Subsystem3 : Subsystem
  Subsystem4 : Subsystem
  Switch : Switch  Criteria=u2 ~= 0
  TOS : Subsystem
  UDP Receive (3)\Data Received : dsmpblib/Hardware-Triggered Runnable Function
      settings: SourceProductName=dSPACE Model Interface Blockset
  UDP Receive 2\Data Received : dsmpblib/Hardware-Triggered Runnable Function
      settings: SourceProductName=dSPACE Model Interface Blockset
  UDP_Received : Subsystem
  Unit Delay : UnitDelay  Commented=on  SampleTime=-1  HasFrameUpgradeWarning=on
  Unit Delay{1..5} (5 alike) : UnitDelay  SampleTime=-1  HasFrameUpgradeWarning=on
  VCANBus : dsmpblib/Data Inport  Priority=10000
      settings: SourceProductName=dSPACE Model Interface Blockset
  aeb : Subsystem  Tag=<DSModel=2_'Osm'>
      settings: AttributesFormatString=<DSModel='Osm'>
  ifLaneBus_out_In : dsmpblib/Data Inport  Priority=10000
      settings: SourceProductName=dSPACE Model Interface Blockset
  wires:
  Subsystem2/1(TOS_ACCP0) -> Rate Transition76/1  "TOS_ACCP0"
  Rate Transition13/1 -> Bus Creator/3  "lanebus"
  Rate Transition61/1 -> Subsystem2/4(visMsg)
  Rate Transition30/1 -> LPV/8(IfVIEBus)
  IfRFM_LANES_In/1 -> Subsystem1/3(lane)
  Rate Transition87/1 -> Rate Transition8/1
  Rate Transition88/1 -> Rate Transition7/1, [LATBus]
  Rate Transition8/1 -> Chassis1/8(IfLonCtrlBus)
  Rate Transition68/1 -> Bus Creator3/8  "TOS_LCKIE"
  Bus Selector2/1 -> Selector1/1, Selector2/1, Selector6/1, Selector3/1  "<EQ4_LA_ELEM>"
  Bus Creator1/1 -> Bus Selector2/1, Bus Selector/1, Rate Transition32/1
  Chassis1/7(ACC_FD2) -> Rate Transition82/1
  Rate Transition46/1 -> IFC_FD3/1
  Rate Transition84/1 -> [ifVSMBus], Rate Transition33/1  "VSM_CTRL_LINE"
  Rate Transition85/1 -> [IfLSMBus]  "VSM_CTRL_LINE"
  EQ4_Lane_Pack1/4(EQ4_LRE) -> Bus Creator1/4  "EQ4_LRE"
  Function-Call Generator5/1 -> Control1/Trigger
  LPV/1(IfVSMBus) -> Rate Transition84/1  "VSM_CTRL_LINE"
  Rate Transition11/1 -> LPV/10(RFM_LANES)
  Rate Transition82/1 -> ACC_FD2/1
  Selector2/1 -> Subsystem4/6(EQ4_LA_ELEM_1)
  Subsystem2/11(TOS_AEB_JAOBJ) -> Rate Transition71/1
  Rate Transition10/1 -> Bus Creator/1
  Rate Transition83/1 -> ACC_FD4/1
  [CSASim_IDC_L2_LampReq] -> Rate Transition28/1
  Rate Transition1/1 -> Chassis1/14(LaneBus)  "lanebus"
  Rate Transition27/1 -> IFC_FD2/1
  UDP_Received/1(visMsg) -> [visMsg]
  Subsystem2/12(TOS_P0_TARGET_LINE) -> Rate Transition75/1
  Subsystem2/13(TOS_UpdateCnt) -> Rate Transition72/1
  Rate Transition69/1 -> Bus Creator3/9  "TOS_AEB_LONOBJ"
  [IfEHRBus] -> Rate Transition36/1
  CAL/1(IfCALBus) -> [IfCALBus]
  Rate Transition72/1 -> Bus Creator3/13  "TOS_UpdateCnt"
  From20/1 -> Rate Transition74/1  "TOS_LC"
  [AEBBus] -> Unit Delay3/1
  Subsystem2/2(TOS_ACCP1) -> Rate Transition77/1
  [IfVIEBus] -> Rate Transition37/1
  Rate Transition66/1 -> Bus Creator3/7  "TOS_ELK"
  [IfCALBus] -> Rate Transition41/1
  Rate Transition18/1 -> Bus Creator/5  "lonbus"
  Rate Transition63/1 -> Bus Creator3/4  "TOS_ACCP3"
  [IfLSMBus] -> Rate Transition17/1
  Rate Transition19/1 -> Control1/1(IfVCANBus)
  Rate Transition73/1 -> Subsystem2/3(IfVCAN)
  Rate Transition76/1 -> Bus Creator3/1  "TOS_ACCP0"
  Rate Transition77/1 -> Bus Creator3/2  "TOS_ACCP1"
  Rate Transition20/1 -> Bus Creator/6  "latbus"
  From27/1 -> Rate Transition73/1
  UDP Receive 2\Data Received/1 -> UDP_Received/Trigger
  Unit Delay/1 -> Rate Transition78/1
  Rate Transition81/1 -> ACC_FD1/1
  From15/1 -> Unit Delay/1
  Rate Transition74/1 -> Bus Creator3/14  "TOS_LC"
  [IfLSMBus] -> Bus Selector1/1
  Chassis1/1(IFC_FD1) -> Rate Transition25/1
  Chassis1/8(ACC_FD4) -> Rate Transition83/1
  Subsystem1/1(IfRFM_LANES_In) -> [RFM_LANES]
  EQ4_Lane_Pack1/3(EQ4_LH) -> Bus Creator1/3  "EQ4_LH"
  [IfCANBus] -> Rate Transition42/1
  Rate Transition22/1 -> LPV/4(IfCANBus)
  Function-Call Generator3/1 -> Common1/Trigger
  Rate Transition32/1 -> LPV/9(IfEQ4Bus)
  [IfLineBus] -> Rate Transition13/1  "lanebus"
  Rate Transition17/1 -> Chassis1/7(IfLSMBus)
  Bus Selector2/2 -> Subsystem4/9(LA_HDR)  "<EQ4_LA_HDR>"
  Rate Transition12/1 -> Bus Creator/2
  Rate Transition15/1 -> Chassis1/10(IfPlanbus)
  [ifVSMBus] -> Rate Transition26/1
  Function-Call Generator1/1 -> Chassis1/Trigger
  Subsystem3/1(Out2) -> Rate Transition21/1
  Rate Transition9/1 -> Control1/8(IfPlanbus)
  Unit Delay3/1 -> Rate Transition39/1  "aebbus"
  Rate Transition28/1 -> Chassis1/18(CSASim_IDC_L2_LampReq)
  EQ4_Lane_Pack1/1(EQ4_LAP) -> Bus Creator1/1  "EQ4_LAP"
  Chassis1/2(IFC_FD2) -> Rate Transition27/1
  Rate Transition34/1 -> Control1/3(IfTOSBus)
  Selector1/1 -> Subsystem4/5(EQ4_LA_ELEM_0)
  Control1/1(IfLONBus) -> [LONBus], Rate Transition87/1
  Rate Transition64/1 -> Bus Creator3/5  "TOS_ACCP4"
  UDP Receive (3)\Data Received/1 -> Subsystem3/Trigger
  Bus Selector2/3 -> Subsystem4/10(In10)  "<EQ4_LRE_ELEM>"
  Chassis1/6(ACC_FD1) -> Rate Transition81/1
  Chassis1/5(IFC_FD6) -> Rate Transition80/1
  Rate Transition86/1 -> Rate Transition9/1, Rate Transition15/1, [ifPlanbus]  "VSM_CTRL_LINE"
  RFM_Road/1 -> Subsystem1/2(RFM_Road)
  CR_RSDS_Input/1(LC_Obj) -> [LC_Obj]
  Rate Transition24/1 -> Control1/9(roadwidth)
  [IfCANBus] -> Rate Transition19/1
  Selector5/1 -> Subsystem4/2(EQ4_LH_ELEM_1)
  Bus Selector/1 -> Selector4/1, Selector5/1  "<EQ4_LH_ELEM>"
  Rate Transition3/1 -> Common1/1(IfCANBus)  "lonbus"
  Rate Transition21/1 -> Subsystem1/1(l3_RFMResult)  "lonbus"
  Rate Transition65/1 -> Bus Creator3/6  "TOS_ACCP5"
  Bus Selector/2 -> Subsystem4/3(LH_HDR)  "<EQ4_LH_HDR>"
  Rate Transition67/1 -> Subsystem2/2(IfVIEBus)
  Unit Delay2/1 -> Rate Transition18/1  "lonbus"
  From14/1 -> Rate Transition67/1
  Control1/2(IfLATBus) -> Rate Transition88/1
  Common1/2(IfDMSBus) -> [IfDMSBus]
  Rate Transition36/1 -> Control1/5(IfEHRBus)
  Common1/3(IfVIEBus) -> [IfVIEBus]
  Rate Transition41/1 -> Chassis1/4(IfCALBus)
  Rate Transition45/1 -> Chassis1/17(RoadBus)  "lanebus"
  Chassis1/4(IFC_FD5) -> Rate Transition79/1
  LPV/3(IfPlanbus) -> Rate Transition86/1
  Common1/4(IfEHRBus) -> [IfEHRBus]
  Rate Transition43/1 -> Chassis1/15(IfAEBBus)  "lanebus"
  [IfCANBus] -> Rate Transition3/1
  [IfLineBus] -> Rate Transition1/1  "lanebus"
  Rate Transition44/1 -> Chassis1/16(IfOSMBus)  "lanebus"
  Rate Transition26/1 -> Chassis1/6(IfVSMBus)
  Rate Transition70/1 -> Bus Creator3/10  "TOS_AEB_LATOBJ"
  [IfEHRBus] -> Rate Transition6/1
  Rate Transition7/1 -> Chassis1/9(IfLatCtrlBus)
  [visMsg] -> Rate Transition31/1
  LPV/2(IfLSMBus) -> Rate Transition85/1
  Selector3/1 -> Subsystem4/7(EQ4_LA_ELEM_2)
  [IfVIEBus] -> Rate Transition40/1
  [RoadBus] -> Rate Transition45/1  "roadbus"
  [visMsg] -> Rate Transition16/1
  Rate Transition80/1 -> IFC_FD6/1
  [LONBus] -> Unit Delay2/1
  [RoadBus] -> Rate Transition14/1  "roadbus"
  Rate Transition33/1 -> Control1/2(IfVSMBus)
  [ifVSMBus] -> aeb/3(IfVSMBus)
  Rate Transition25/1 -> IFC_FD1/1
  Rate Transition35/1 -> Control1/4(IfRFMBus)
  Bus Creator/1 -> LPV/3(IfALLBus)
  Rate Transition23/1 -> LPV/6(IfDMSBus)
  aeb/1(IfAEBSBus) -> Rate Transition43/1, [AEBBus]
  [IfVIEBus] -> aeb/2(IfVIEBus)
  [LATBus] -> Unit Delay1/1
  [RoadBus] -> Rate Transition38/1
  Rate Transition5/1 -> LPV/5(IfCALBus)
  Subsystem2/6(TOS_ACCP5) -> Rate Transition65/1
  Bus Selector1/1 -> Rate Transition24/1  "<RoadWidth>"
  Function-Call Generator4/1 -> LPV/Trigger
  [IfVIEBus] -> Rate Transition30/1
  Chassis1/3(IFC_FD3) -> Rate Transition46/1
  [IfDMSBus] -> Rate Transition23/1
  Selector6/1 -> Subsystem4/8(EQ4_LA_ELEM_3)
  [IfCANBus] -> Rate Transition22/1
  [RFM_LANES] -> Rate Transition11/1
  Rate Transition16/1 -> Chassis1/11(IfVEQ4Bus)
  Rate Transition39/1 -> Bus Creator/7  "aebbus"
  Rate Transition40/1 -> Chassis1/5(IfVIEBus)
  Rate Transition71/1 -> Bus Creator3/11  "TOS_AEB_JAOBJ"
  Selector4/1 -> Subsystem4/1(EQ4_LH_ELEM_0)
  [IfEHRBus] -> Rate Transition29/1
  Subsystem2/3(ACCP2) -> Rate Transition62/1
  Unit Delay1/1 -> Rate Transition20/1  "latbus"
  [IfCALBus] -> Rate Transition5/1
  From21/1 -> Rate Transition61/1
  Software-Triggered Runnable Function/1 -> Subsystem2/Trigger
  EQ4_Lane_Pack1/2(EQ4_LA) -> Bus Creator1/2  "EQ4_LA"
  ifLaneBus_out_In/1 -> Subsystem4/4(lanebus)  "lanebus"
  Subsystem2/10(TOS_AEB_LATOBJ) -> Rate Transition70/1
  Rate Transition37/1 -> Control1/6(IfVIEBus)
  Rate Transition79/1 -> IFC_FD5/1
  Rate Transition31/1 -> EQ4_Lane_Pack1/1(In1)  "visMsg"
  Subsystem2/4(ACCP3) -> Rate Transition63/1
  Rate Transition38/1 -> Control1/7(IfRoadBus)
  Subsystem2/9(TOS_AEB_LONOBJ) -> Rate Transition69/1
  Rate Transition29/1 -> LPV/7(IfEHRBus)
  [IfDMSBus] -> Rate Transition4/1
  Subsystem2/8(TOS_LCKIE) -> Rate Transition68/1
  Rate Transition4/1 -> Chassis1/13(IfDMSBus)
  Rate Transition14/1 -> Bus Creator/4  "roadbus"
  Subsystem4/1(Out1) -> [IfLineBus]
  Rate Transition62/1 -> Bus Creator3/3  "TOS_ACCP2"
  Subsystem1/2(roadbus) -> [RoadBus]  "roadbus"
  [IfLineBus] -> Rate Transition35/1
  Subsystem2/7(TOS_ELK) -> Rate Transition66/1
  [ifObjectBus] -> Rate Transition12/1
  Rate Transition6/1 -> Chassis1/12(IfEHRBus)
  Subsystem2/5(TOS_ACCP4) -> Rate Transition64/1
  Rate Transition42/1 -> Chassis1/3(IfVCANBus)
  Rate Transition78/1 -> Subsystem2/1(IfStateMBus)
  Rate Transition75/1 -> Bus Creator3/12  "TOS_P0_TARGET_LINE"
  Constant13/1 -> Switch/2
  Bus Assignment1/1 -> Switch/1
  SimBCM/2(RTurnLmpSwtSts) -> Rate Transition92/1
  SimBCM/1(LTurnLmpSwtSts) -> Rate Transition91/1
  Rate Transition90/1 -> SimBCM/1(VCAN)
  Function-Call Generator2/1 -> SimBCM/Trigger
  Rate Transition91/1 -> Bus Assignment1/2
  Rate Transition92/1 -> Bus Assignment1/3
  Rate Transition89/1 -> Unit Delay5/1
  Unit Delay5/1 -> SimBCM/2(PLAN_ALC_DECS)
  VCANBus/1 -> Rate Transition90/1, Bus Assignment1/1, Switch/3
  [ifPlanbus] -> Rate Transition89/1
  SimBCM/3(CSASim_IDC_L2_LampReq) -> [CSASim_IDC_L2_LampReq]
  Switch/1 -> [IfCANBus]
  [LC_Obj] -> TOS/5(LC_Obj)
  [visMsg] -> TOS/4(VisMsg)
  [IfCANBus] -> TOS/3(IfVCAN)
  [IfVIEBus] -> TOS/2(IfVIEBus)
  Unit Delay4/1 -> TOS/1(IfStateMBus)
  [ifVSMBus] -> Unit Delay4/1
  TOS/1(IfTOSBus) -> Rate Transition44/1, Rate Transition34/1, Rate Transition10/1
